simulink model "FullFMS_2025_12_15_V0_3_7"  (R2025b)
settings: Solver=ode23tb  StartTime=0.0  StopTime=inf  MaxStep=0.1  RelTol=1e-2
PreLoadFcn:
  | load("BUS_CONFIG.mat")
libraries: opcualib x8
(part 1 of 4)
settings Model: SimulationMode=accelerator  PacingRate=0.100000  Creator=guilh  LastModifiedBy=vitor
settings SolverCC: ZeroCrossControl=DisableAll

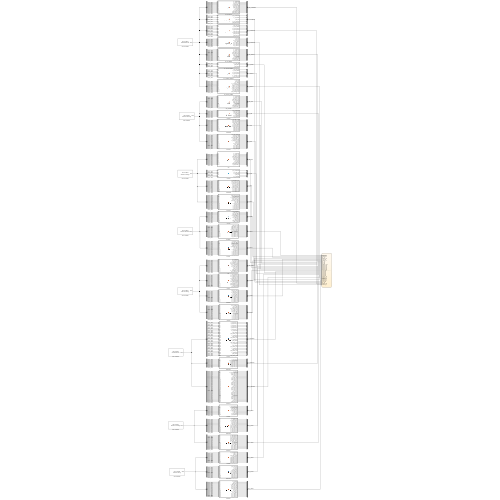
[thumbnail: Simulink's stored preview of the top-level diagram]
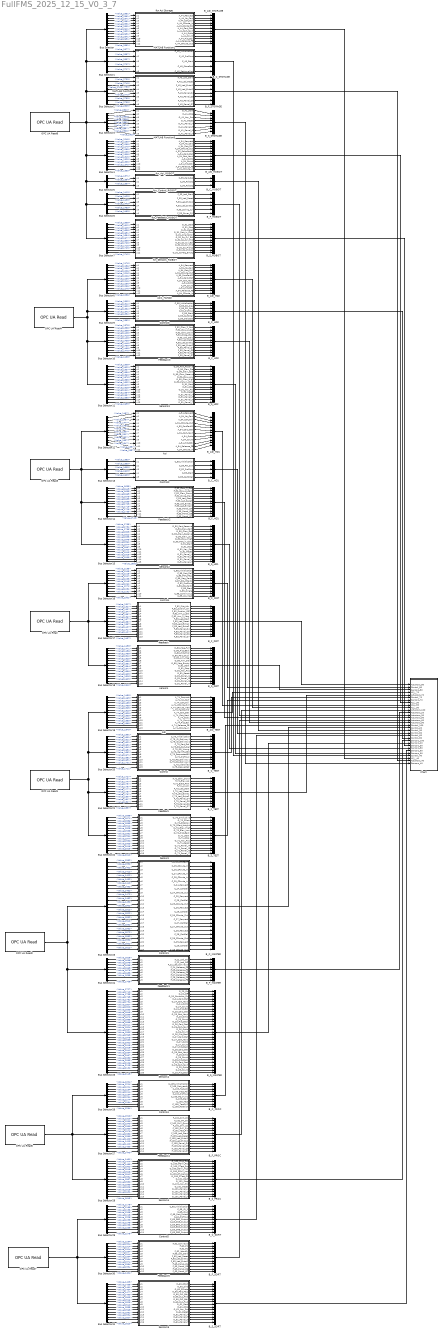
== system FullFMS_2025_12_15_V0_3_7 ==
  ASI : MATLAB Function  TreatAsAtomicUnit=on
  Asi : MATLAB Function  TreatAsAtomicUnit=on
  Asi1_HAND2 : MATLAB Function  TreatAsAtomicUnit=on
  B_ASI_HD1 : BusCreator  Inputs=12  OutDataTypeStr=Bus: B_ASI_HD1  NonVirtualBus=on
  B_ASI_HD2 : BusCreator  Inputs=12  OutDataTypeStr=Bus: B_ASI_HD2  NonVirtualBus=on
  B_ASI_ROBOT : BusCreator  Inputs=12  OutDataTypeStr=Bus: B_ASI_ROBOT  NonVirtualBus=on
  B_ASI_STORAGE : BusCreator  Inputs=12  OutDataTypeStr=Bus: B_ASI_STORAGE  NonVirtualBus=on
  B_ASI_TEST : BusCreator  Inputs=13  OutDataTypeStr=Bus: B_ASI_TEST  NonVirtualBus=on
  B_C_DIST : BusCreator  Inputs=11  OutDataTypeStr=Bus: B_C_DIST  NonVirtualBus=on
  B_C_HD1 : BusCreator  Inputs=5  OutDataTypeStr=Bus: B_C_HD1  NonVirtualBus=on
  B_C_HD2 : BusCreator  Inputs=7  OutDataTypeStr=Bus: B_C_HD2  NonVirtualBus=on
  B_C_MASTER : BusCreator  Inputs=24  OutDataTypeStr=Bus: B_C_MASTER  NonVirtualBus=on
  B_C_PROC : BusCreator  Inputs=10  OutDataTypeStr=Bus: B_C_PROC  NonVirtualBus=on
  B_C_ROBOT : BusCreator  Inputs=3  OutDataTypeStr=Bus: B_C_ROBOT  NonVirtualBus=on
  B_C_SORT : BusCreator  Inputs=11  OutDataTypeStr=Bus: B_C_SORT  NonVirtualBus=on
  B_C_STORAGE : BusCreator  Inputs=5  OutDataTypeStr=Bus: B_C_STORAGE  NonVirtualBus=on
  B_C_TEST : BusCreator  Inputs=13  OutDataTypeStr=Bus: B_C_TEST  NonVirtualBus=on
  B_F_DIST : BusCreator  Inputs=13  OutDataTypeStr=Bus: B_F_DIST  NonVirtualBus=on
  B_F_HD1 : BusCreator  Inputs=12  OutDataTypeStr=Bus: B_F_HD1  NonVirtualBus=on
  B_F_HD2 : BusCreator  Inputs=12  OutDataTypeStr=Bus: B_F_HD2  NonVirtualBus=on
  B_F_MASTER : BusCreator  Inputs=9  OutDataTypeStr=Bus: B_F_MASTER  NonVirtualBus=on
  B_F_PROC : BusCreator  Inputs=14  OutDataTypeStr=Bus: B_F_PROC  NonVirtualBus=on
  B_F_ROBOT : BusCreator  Inputs=6  OutDataTypeStr=Bus: B_F_ROBOT  NonVirtualBus=on
  B_F_SORT : BusCreator  Inputs=12  OutDataTypeStr=Bus: B_F_SORT  NonVirtualBus=on
  B_F_STORAGE : BusCreator  Inputs=8  OutDataTypeStr=Bus: B_F_STORAGE  NonVirtualBus=on
  B_F_TEST : BusCreator  Inputs=12  OutDataTypeStr=Bus: B_F_TEST  NonVirtualBus=on
  B_S_DIST : BusCreator  Inputs=15  OutDataTypeStr=Bus: B_S_DIST  NonVirtualBus=on
  B_S_HD1 : BusCreator  Inputs=15  OutDataTypeStr=Bus: B_S_HD1  NonVirtualBus=on
  B_S_HD2 : BusCreator  Inputs=15  OutDataTypeStr=Bus: B_S_HD2  NonVirtualBus=on
  B_S_MASTER : BusCreator  Inputs=33  OutDataTypeStr=Bus: B_S_MASTER  NonVirtualBus=on
  B_S_PROC : BusCreator  Inputs=15  OutDataTypeStr=Bus: B_S_PROC  NonVirtualBus=on
  B_S_ROBOT : BusCreator  Inputs=12  OutDataTypeStr=Bus: B_S_ROBOT  NonVirtualBus=on
  B_S_SORT : BusCreator  Inputs=16  OutDataTypeStr=Bus: B_S_SORT  NonVirtualBus=on
  B_S_STORAGE : BusCreator  Inputs=8  OutDataTypeStr=Bus: B_S_STORAGE  NonVirtualBus=on
  B_S_TEST : BusCreator  Inputs=15  OutDataTypeStr=Bus: B_S_TEST  NonVirtualBus=on
  Bus Selector : BusSelector  OutputSignals=Value_2551,Value_2561,Value_2571,Value_2581,Value_2591,Value_2601,Value_2611,Value_2621,Value_2631,Value_2641,Value_2651,Value_2661
  Bus Selector1 : BusSelector  OutputSignals=Value_2677,Value_2687,Value_2697,Value_2707,Value_2717
  Bus Selector10 : BusSelector  OutputSignals=Value_1378,Value_1388,Value_1398,Value_1408,Value_1418,Value_1428,Value_1438,Value_1448,Value_1458,Value_1468,Value_1478,Value_1488
  Bus Selector11 : BusSelector  OutputSignals=Value_1509,Value_1522,Value_1537,Value_1550,Value_1563,Value_1576,Value_1589,Value_1602,Value_1615,Value_1628,Value_1641,Value_1654,Value_1667,Value_1680,Value_1693
  Bus Selector12 : BusSelector  OutputSignals=Value_1457,Value_1467,Value_1477,Value_1487,Value_1497,Value_1507,Value_1517,Value_1527,Value_1537,Value_1547,Value_1557,Value_1567
  Bus Selector13 : BusSelector  OutputSignals=Value_1583,Value_1593,Value_1603,Value_1613,Value_1623
  Bus Selector14 : BusSelector  OutputSignals=Value_1639,Value_1649,Value_1659,Value_1669,Value_1679,Value_1689,Value_1699,Value_1709,Value_1719,Value_1729,Value_1739,Value_1749
  Bus Selector15 : BusSelector  OutputSignals=Value_1768,Value_1781,Value_1796,Value_1809,Value_1822,Value_1835,Value_1848,Value_1861,Value_1874,Value_1887,Value_1900,Value_1913,Value_1926,Value_1939,Value_1952
  Bus Selector16 : BusSelector  OutputSignals=Value_1195,Value_1205,Value_1215,Value_1227,Value_1239,Value_1249,Value_1261,Value_1271,Value_1281,Value_1291,Value_1301
  Bus Selector17 : BusSelector  OutputSignals=Value_1317,Value_1327,Value_1337,Value_1347,Value_1357,Value_1367,Value_1377,Value_1387,Value_1397,Value_1407,Value_1417,Value_1427,Value_1437
  Bus Selector18 : BusSelector  OutputSignals=Value_1458,Value_1471,Value_1486,Value_1499,Value_1512,Value_1525,Value_1538,Value_1551,Value_1564,Value_1577,Value_1590,Value_1603,Value_1616,Value_1629,Value_1642
  Bus Selector19 : BusSelector  OutputSignals=Value_1455,Value_1465,Value_1475,Value_1485,Value_1495,Value_1505,Value_1515,Value_1525,Value_1535,Value_1545,Value_1555,Value_1565,Value_1575
  Bus Selector2 : BusSelector  OutputSignals=Value_2733,Value_2743,Value_2753,Value_2763,Value_2773,Value_2783,Value_2793,Value_2803
  Bus Selector20 : BusSelector  OutputSignals=Value_1591,Value_1601,Value_1611,Value_1621,Value_1631,Value_1641,Value_1651,Value_1661,Value_1671,Value_1681,Value_1691,Value_1701,Value_1711
  Bus Selector21 : BusSelector  OutputSignals=Value_1727,Value_1737,Value_1747,Value_1757,Value_1767,Value_1777,Value_1787,Value_1797,Value_1807,Value_1817,Value_1827,Value_1837
  Bus Selector22 : BusSelector  OutputSignals=Value_1858,Value_1871,Value_1886,Value_1899,Value_1912,Value_1925,Value_1938,Value_1951,Value_1964,Value_1977,Value_1990,Value_2003,Value_2016,Value_2029,Value_2042
  Bus Selector23 : BusSelector  OutputSignals=Value_1382,Value_1392,Value_1402,Value_1412,Value_1422,Value_1432,Value_1442,Value_1452,Value_1462,Value_1472,Value_1482,Value_1492,Value_1502,Value_1512,Value_1522,Value_1532,Value_1542,Value_1552,Value_1562,Value_1572,Value_1582,Value_1592,Value_1602,Value_1612
  Bus Selector24 : BusSelector  OutputSignals=Value_1628,Value_1638,Value_1648,Value_1658,Value_1668,Value_1678,Value_1688,Value_1698,Value_1708
  Bus Selector25 : BusSelector  OutputSignals=Value_1727,Value_1740,Value_1755,Value_1768,Value_1781,Value_1794,Value_1807,Value_1820,Value_1833,Value_1846,Value_1859,Value_1872,Value_1885,Value_1898,Value_1911,Value_1924,Value_1937,Value_1950,Value_1963,Value_1976,Value_1989,Value_2002,Value_2015,Value_2028,Value_2041,Value_2054,Value_2067,Value_2080,Value_2093,Value_2106,Value_2119,Value_2132,Value_2145
  Bus Selector26 : BusSelector  OutputSignals=Value_1204,Value_1214,Value_1224,Value_1234,Value_1244,Value_1254,Value_1264,Value_1274,Value_1284,Value_1294
  Bus Selector27 : BusSelector  OutputSignals=Value_1310,Value_1320,Value_1330,Value_1340,Value_1350,Value_1360,Value_1370,Value_1380,Value_1390,Value_1400,Value_1410,Value_1420,Value_1430,Value_1440
  Bus Selector28 : BusSelector  OutputSignals=Value_1461,Value_1474,Value_1489,Value_1502,Value_1515,Value_1528,Value_1541,Value_1554,Value_1567,Value_1580,Value_1593,Value_1606,Value_1619,Value_1632,Value_1645
  Bus Selector29 : BusSelector  OutputSignals=Value_1178,Value_1188,Value_1198,Value_1208,Value_1218,Value_1228,Value_1238,Value_1248,Value_1258,Value_1268,Value_1278
  Bus Selector3 : BusSelector  OutputSignals=Value_2822,Value_2835,Value_2848,Value_2861,Value_2874,Value_2887,Value_2900,Value_2913
  Bus Selector30 : BusSelector  OutputSignals=Value_1294,Value_1304,Value_1314,Value_1324,Value_1334,Value_1344,Value_1354,Value_1364,Value_1374,Value_1384,Value_1394,Value_1404
  Bus Selector31 : BusSelector  OutputSignals=Value_1423,Value_1436,Value_1451,Value_1464,Value_1477,Value_1490,Value_1503,Value_1516,Value_1529,Value_1542,Value_1555,Value_1568,Value_1581,Value_1594,Value_1607,Value_1620
  Bus Selector4 : BusSelector  OutputSignals=Value_1245,Value_1255,Value_1265,Value_1275,Value_1285,Value_1295,Value_1305,Value_1315,Value_1325,Value_1335,Value_1345,Value_1355
  Bus Selector5 : BusSelector  OutputSignals=Value_1371,Value_1384,Value_1397
  Bus Selector6 : BusSelector  OutputSignals=Value_1413,Value_1423,Value_1433,Value_1443,Value_1453,Value_1463
  Bus Selector7 : BusSelector  OutputSignals=Value_1599,Value_1612,Value_1625,Value_1638,Value_1651,Value_1664,Value_1677,Value_1690,Value_1703,Value_1716,Value_1729,Value_1742
  Bus Selector8 : BusSelector  OutputSignals=Value_1176,Value_1186,Value_1196,Value_1206,Value_1216,Value_1226,Value_1236,Value_1246,Value_1256,Value_1266,Value_1276,Value_1286
  Bus Selector9 : BusSelector  OutputSignals=Value_1302,Value_1312,Value_1322,Value_1332,Value_1342,Value_1352,Value_1362
  Chart : Stateflow chart  TreatAsAtomicUnit=on
      settings: PortSchema="{\"entries\":[{\"content\":{\"sides\":[{\"content\":{\"connectorIds\":[\"In2\",\"In1\",\"In3\",\"In4\",\"In6\",\"In5\",\"In7\",\"In8\",\"In9\",\"In10\",\"In11\",\"In12\",\"In13\",\"In14\",\"In15\",\"In16\",\"In17\",\"In18\",\"In19\",\"In20\",\"In21\",\"In22\",\"In23\",\"In24\",\"In25\",\"In26\",\"In27\",\"In28\",\"In29\",\"In30\",\"In31\",\"In32\"]},\"type\":\"ConnectorPlacement.EquallySpacedRectSide\",\"uuid\":\"e54bf7d4-7c7d-41d9-a8b8-f479ac319a99\"},{\"content\":{\"side\":\"RIGHT\"},\"type\":\"ConnectorPlacement.EquallySpacedRectSide\",\"uuid\":\"d3c20706-71bd-4e26-b40f-0ee7e71b06ee\"},{\"content\":{\"side\":\"TOP\"},\"type\":\"ConnectorPlacement.EquallySpacedRectSide\",\"uuid\":\"ecfb6920-e95b-4ed8-99f9-df5ce878328e\"}]},\"type\":\"ConnectorPlacement.EquallySpacedConnector\",\"uuid\":\"2e714192-4eea-4e1a-8945-7c827feed48f\"}],\"packageUris\":[\"http://schema.mathworks.com/mf0/Connector/R2020b\"],\"version\":\"1.0\"}"
  Control : MATLAB Function  TreatAsAtomicUnit=on
  Control1 : MATLAB Function  TreatAsAtomicUnit=on
  Control2 : MATLAB Function  TreatAsAtomicUnit=on
  Control3 : MATLAB Function  TreatAsAtomicUnit=on
  Control4 : MATLAB Function  TreatAsAtomicUnit=on
  Control5 : MATLAB Function  TreatAsAtomicUnit=on
  Feedback : MATLAB Function  TreatAsAtomicUnit=on
  Feedback1 : MATLAB Function  TreatAsAtomicUnit=on
  Feedback2 : MATLAB Function  TreatAsAtomicUnit=on
  Feedback3 : MATLAB Function  TreatAsAtomicUnit=on
  Feedback4 : MATLAB Function  TreatAsAtomicUnit=on
  Feedback5 : MATLAB Function  TreatAsAtomicUnit=on
  MATLAB Function1 : MATLAB Function  TreatAsAtomicUnit=on
  MATLAB Function2 : MATLAB Function  TreatAsAtomicUnit=on
  MATLAB Function3 : MATLAB Function  TreatAsAtomicUnit=on
  OPC UA Read : opcualib/OPC UA Read  SelectedServer=AAS OPC Distribution  ServerList=AAS OPC Distribution  NodeList={ '1', 'Value', '6', '1195', '1'; '2', 'Value', '6', '1205', '1'; '3', 'Value', '6', '1215', '1'; '4', 'Value', '6', '1227', '1'; '5', 'Value', '6', '1239', '1'; '6', 'Value', '6', '1249', '1'; '7', 'Value', '6', '1261', '1'; '8', 'Value', '6', '1271', '1'; '9', 'Value', '6', '1281', '1'; '10', 'Value', '6', '1291', '1'; '11', 'Value', '6', '1301', '1'; '12', 'Value', '6', '1317', '1'; '13', 'Value', '6', '1327', '1'; '14', 'Value', '6', '1337', '1'; '15', 'Value', '6', '1347', '1'; '16', 'Value', '6', '1357', '1'; '17', 'Value', '6', '1367', '1'; '18', 'Value', '6', '1377', '1'; '19', 'Value', '6', '1387', '1'; '20', 'Value', '6', '1397', '1'; '21', 'Value', '6', '1407', '1'; '22', 'Value', '6', '1417', '1'; '23', 'Value', '6', '1427', '1'; '24', 'Value', '6', '1437', '1'; '25', 'Value', '6', '1458', '1'; '26', 'Value', '6', '1471', '1'; '27', 'Value', '6', '1486', '1'; '28', 'Value', '6', '1499', '1'; '29', 'Value', '6', '1512', '1'; '30', 'Value', '6', '1525', '1'; '31', 'Value', '6', '1538', '1'; '32', 'Value', '6', '1551', '1'; '33', 'Value', '6', '1564', '1'; '34', 'Value', '6', '1577', '1'; '35', 'Value', '6', '1590', '1'; '36', 'Value', '6', '1603', '1'; '37', 'Value', '6', '1616', '1'; '38', 'Value', '6', '1629', '1'; '39', 'Value', '6', '1642', '1' }  ShowQualityPort=off  ShowTimestampPort=off  ShowTimestampPortAs=Seconds since start  SampleTime=-1
  OPC UA Read1 : opcualib/OPC UA Read  SelectedServer=AAS OPC Testing  ServerList=AAS OPC Testing  NodeList={ '1', 'Value', '6', '1455', '1'; '2', 'Value', '6', '1465', '1'; '3', 'Value', '6', '1475', '1'; '4', 'Value', '6', '1485', '1'; '5', 'Value', '6', '1495', '1'; '6', 'Value', '6', '1505', '1'; '7', 'Value', '6', '1515', '1'; '8', 'Value', '6', '1525', '1'; '9', 'Value', '6', '1535', '1'; '10', 'Value', '6', '1545', '1'; '11', 'Value', '6', '1555', '1'; '12', 'Value', '6', '1565', '1'; '13', 'Value', '6', '1575', '1'; '14', 'Value', '6', '1591', '1'; '15', 'Value', '6', '1601', '1'; '16', 'Value', '6', '1611', '1'; '17', 'Value', '6', '1621', '1'; '18', 'Value', '6', '1631', '1'; '19', 'Value', '6', '1641', '1'; '20', 'Value', '6', '1651', '1'; '21', 'Value', '6', '1661', '1'; '22', 'Value', '6', '1671', '1'; '23', 'Value', '6', '1681', '1'; '24', 'Value', '6', '1691', '1'; '25', 'Value', '6', '1701', '1'; '26', 'Value', '6', '1711', '1'; '27', 'Value', '6', '1727', '1'; '28', 'Value', '6', '1737', '1'; '29', 'Value', '6', '1747', '1'; '30', 'Value', '6', '1757', '1'; '31', 'Value', '6', '1767', '1'; '32', 'Value', '6', '1777', '1'; '33', 'Value', '6', '1787', '1'; '34', 'Value', '6', '1797', '1'; '35', 'Value', '6', '1807', '1'; '36', 'Value', '6', '1817', '1'; '37', 'Value', '6', '1827', '1'; '38', 'Value', '6', '1837', '1'; '39', 'Value', '6', '1858', '1'; '40', 'Value', '6', '1871', '1'; '41', 'Value', '6', '1886', '1'; '42', 'Value', '6', '1899', '1'; '43', 'Value', '6', '1912', '1'; '44', 'Value', '6', '1925', '1'; '45', 'Value', '6', '1938', '1'; '46', 'Value', '6', '1951', '1'; '47', 'Value', '6', '1964', '1'; '48', 'Value', '6', '1977', '1'; '49', 'Value', '6', '1990', '1'; '50', 'Value', '6', '2003', '1'; '51', 'Value', '6', '2016', '1'; '52', 'Value', '6', '2029', '1'; '53', 'Value', '6', '2042', '1' }  ShowQualityPort=off  ShowTimestampPort=off  ShowTimestampPortAs=Seconds since start  SampleTime=-1
  OPC UA Read2 : opcualib/OPC UA Read  SelectedServer=AAS OPC Master  ServerList=AAS OPC Master  NodeList={ '1', 'Value', '6', '1382', '1'; '2', 'Value', '6', '1392', '1'; '3', 'Value', '6', '1402', '1'; '4', 'Value', '6', '1412', '1'; '5', 'Value', '6', '1422', '1'; '6', 'Value', '6', '1432', '1'; '7', 'Value', '6', '1442', '1'; '8', 'Value', '6', '1452', '1'; '9', 'Value', '6', '1462', '1'; '10', 'Value', '6', '1472', '1'; '11', 'Value', '6', '1482', '1'; '12', 'Value', '6', '1492', '1'; '13', 'Value', '6', '1502', '1'; '14', 'Value', '6', '1512', '1'; '15', 'Value', '6', '1522', '1'; '16', 'Value', '6', '1532', '1'; '17', 'Value', '6', '1542', '1'; '18', 'Value', '6', '1552', '1'; '19', 'Value', '6', '1562', '1'; '20', 'Value', '6', '1572', '1'; '21', 'Value', '6', '1582', '1'; '22', 'Value', '6', '1592', '1'; '23', 'Value', '6', '1602', '1'; '24', 'Value', '6', '1612', '1'; '25', 'Value', '6', '1628', '1'; '26', 'Value', '6', '1638', '1'; '27', 'Value', '6', '1648', '1'; '28', 'Value', '6', '1658', '1'; '29', 'Value', '6', '1668', '1'; '30', 'Value', '6', '1678', '1'; '31', 'Value', '6', '1688', '1'; '32', 'Value', '6', '1698', '1'; '33', 'Value', '6', '1708', '1'; '34', 'Value', '6', '1727', '1'; '35', 'Value', '6', '1740', '1'; '36', 'Value', '6', '1755', '1'; '37', 'Value', '6', '1768', '1'; '38', 'Value', '6', '1781', '1'; '39', 'Value', '6', '1794', '1'; '40', 'Value', '6', '1807', '1'; '41', 'Value', '6', '1820', '1'; '42', 'Value', '6', '1833', '1'; '43', 'Value', '6', '1846', '1'; '44', 'Value', '6', '1859', '1'; '45', 'Value', '6', '1872', '1'; '46', 'Value', '6', '1885', '1'; '47', 'Value', '6', '1898', '1'; '48', 'Value', '6', '1911', '1'; '49', 'Value', '6', '1924', '1'; '50', 'Value', '6', '1937', '1'; '51', 'Value', '6', '1950', '1'; '52', 'Value', '6', '1963', '1'; '53', 'Value', '6', '1976', '1'; '54', 'Value', '6', '1989', '1'; '55', 'Value', '6', '2002', '1'; '56', 'Value', '6', '2015', '1'; '57', 'Value', '6', '2028', '1'; '58', 'Value', '6', '2041', '1'; '59', 'Value', '6', '2054', '1'; '60', 'Value', '6', '2067', '1'; '61', 'Value', '6', '2080', '1'; '62', 'Value', '6', '2093', '1'; '63', 'Value', '6', '2106', '1'; '64', 'Value', '6', '2119', '1'; '65', 'Value', '6', '2132', '1'; '66', 'Value', '6', '2145', '1' }  ShowQualityPort=off  ShowTimestampPort=off  ShowTimestampPortAs=Seconds since start  SampleTime=-1
  OPC UA Read3 : opcualib/OPC UA Read  SelectedServer=AAS OPC Handling1  ServerList=AAS OPC Handling1  NodeList={ '1', 'Value', '6', '1457', '1'; '2', 'Value', '6', '1467', '1'; '3', 'Value', '6', '1477', '1'; '4', 'Value', '6', '1487', '1'; '5', 'Value', '6', '1497', '1'; '6', 'Value', '6', '1507', '1'; '7', 'Value', '6', '1517', '1'; '8', 'Value', '6', '1527', '1'; '9', 'Value', '6', '1537', '1'; '10', 'Value', '6', '1547', '1'; '11', 'Value', '6', '1557', '1'; '12', 'Value', '6', '1567', '1'; '13', 'Value', '6', '1583', '1'; '14', 'Value', '6', '1593', '1'; '15', 'Value', '6', '1603', '1'; '16', 'Value', '6', '1613', '1'; '17', 'Value', '6', '1623', '1'; '18', 'Value', '6', '1639', '1'; '19', 'Value', '6', '1649', '1'; '20', 'Value', '6', '1659', '1'; '21', 'Value', '6', '1669', '1'; '22', 'Value', '6', '1679', '1'; '23', 'Value', '6', '1689', '1'; '24', 'Value', '6', '1699', '1'; '25', 'Value', '6', '1709', '1'; '26', 'Value', '6', '1719', '1'; '27', 'Value', '6', '1729', '1'; '28', 'Value', '6', '1739', '1'; '29', 'Value', '6', '1749', '1'; '30', 'Value', '6', '1768', '1'; '31', 'Value', '6', '1781', '1'; '32', 'Value', '6', '1796', '1'; '33', 'Value', '6', '1809', '1'; '34', 'Value', '6', '1822', '1'; '35', 'Value', '6', '1835', '1'; '36', 'Value', '6', '1848', '1'; '37', 'Value', '6', '1861', '1'; '38', 'Value', '6', '1874', '1'; '39', 'Value', '6', '1887', '1'; '40', 'Value', '6', '1900', '1'; '41', 'Value', '6', '1913', '1'; '42', 'Value', '6', '1926', '1'; '43', 'Value', '6', '1939', '1'; '44', 'Value', '6', '1952', '1' }  ShowQualityPort=off  ShowTimestampPort=off  ShowTimestampPortAs=Seconds since start  SampleTime=-1
  OPC UA Read4 : opcualib/OPC UA Read  SelectedServer=AAS OPC Handling2  ServerList=AAS OPC Handling2  NodeList={ '1', 'Value', '6', '1176', '1'; '2', 'Value', '6', '1186', '1'; '3', 'Value', '6', '1196', '1'; '4', 'Value', '6', '1206', '1'; '5', 'Value', '6', '1216', '1'; '6', 'Value', '6', '1226', '1'; '7', 'Value', '6', '1236', '1'; '8', 'Value', '6', '1246', '1'; '9', 'Value', '6', '1256', '1'; '10', 'Value', '6', '1266', '1'; '11', 'Value', '6', '1276', '1'; '12', 'Value', '6', '1286', '1'; '13', 'Value', '6', '1302', '1'; '14', 'Value', '6', '1312', '1'; '15', 'Value', '6', '1322', '1'; '16', 'Value', '6', '1332', '1'; '17', 'Value', '6', '1342', '1'; '18', 'Value', '6', '1352', '1'; '19', 'Value', '6', '1362', '1'; '20', 'Value', '6', '1378', '1'; '21', 'Value', '6', '1388', '1'; '22', 'Value', '6', '1398', '1'; '23', 'Value', '6', '1408', '1'; '24', 'Value', '6', '1418', '1'; '25', 'Value', '6', '1428', '1'; '26', 'Value', '6', '1438', '1'; '27', 'Value', '6', '1448', '1'; '28', 'Value', '6', '1458', '1'; '29', 'Value', '6', '1468', '1'; '30', 'Value', '6', '1478', '1'; '31', 'Value', '6', '1488', '1'; '32', 'Value', '6', '1509', '1'; '33', 'Value', '6', '1522', '1'; '34', 'Value', '6', '1537', '1'; '35', 'Value', '6', '1550', '1'; '36', 'Value', '6', '1563', '1'; '37', 'Value', '6', '1576', '1'; '38', 'Value', '6', '1589', '1'; '39', 'Value', '6', '1602', '1'; '40', 'Value', '6', '1615', '1'; '41', 'Value', '6', '1628', '1'; '42', 'Value', '6', '1641', '1'; '43', 'Value', '6', '1654', '1'; '44', 'Value', '6', '1667', '1'; '45', 'Value', '6', '1680', '1'; '46', 'Value', '6', '1693', '1' }  ShowQualityPort=off  ShowTimestampPort=off  ShowTimestampPortAs=Seconds since start  SampleTime=-1
  OPC UA Read5 : opcualib/OPC UA Read  SelectedServer=AAS OPC Processing  ServerList=AAS OPC Processing  NodeList={ '1', 'Value', '6', '1204', '1'; '2', 'Value', '6', '1214', '1'; '3', 'Value', '6', '1224', '1'; '4', 'Value', '6', '1234', '1'; '5', 'Value', '6', '1244', '1'; '6', 'Value', '6', '1254', '1'; '7', 'Value', '6', '1264', '1'; '8', 'Value', '6', '1274', '1'; '9', 'Value', '6', '1284', '1'; '10', 'Value', '6', '1294', '1'; '11', 'Value', '6', '1310', '1'; '12', 'Value', '6', '1320', '1'; '13', 'Value', '6', '1330', '1'; '14', 'Value', '6', '1340', '1'; '15', 'Value', '6', '1350', '1'; '16', 'Value', '6', '1360', '1'; '17', 'Value', '6', '1370', '1'; '18', 'Value', '6', '1380', '1'; '19', 'Value', '6', '1390', '1'; '20', 'Value', '6', '1400', '1'; '21', 'Value', '6', '1410', '1'; '22', 'Value', '6', '1420', '1'; '23', 'Value', '6', '1430', '1'; '24', 'Value', '6', '1440', '1'; '25', 'Value', '6', '1461', '1'; '26', 'Value', '6', '1474', '1'; '27', 'Value', '6', '1489', '1'; '28', 'Value', '6', '1502', '1'; '29', 'Value', '6', '1515', '1'; '30', 'Value', '6', '1528', '1'; '31', 'Value', '6', '1541', '1'; '32', 'Value', '6', '1554', '1'; '33', 'Value', '6', '1567', '1'; '34', 'Value', '6', '1580', '1'; '35', 'Value', '6', '1593', '1'; '36', 'Value', '6', '1606', '1'; '37', 'Value', '6', '1619', '1'; '38', 'Value', '6', '1632', '1'; '39', 'Value', '6', '1645', '1' }  ShowQualityPort=off  ShowTimestampPort=off  ShowTimestampPortAs=Seconds since start  SampleTime=-1
  OPC UA Read6 : opcualib/OPC UA Read  SelectedServer=Node-RED OPCUA  ServerList=Node-RED OPCUA  NodeList={ '1', 'Value', '6', '2551', '1'; '2', 'Value', '6', '2561', '1'; '3', 'Value', '6', '2571', '1'; '4', 'Value', '6', '2581', '1'; '5', 'Value', '6', '2591', '1'; '6', 'Value', '6', '2601', '1'; '7', 'Value', '6', '2611', '1'; '8', 'Value', '6', '2621', '1'; '9', 'Value', '6', '2631', '1'; '10', 'Value', '6', '2641', '1'; '11', 'Value', '6', '2651', '1'; '12', 'Value', '6', '2661', '1'; '13', 'Value', '6', '2677', '1'; '14', 'Value', '6', '2687', '1'; '15', 'Value', '6', '2697', '1'; '16', 'Value', '6', '2707', '1'; '17', 'Value', '6', '2717', '1'; '18', 'Value', '6', '2733', '1'; '19', 'Value', '6', '2743', '1'; '20', 'Value', '6', '2753', '1'; '21', 'Value', '6', '2763', '1'; '22', 'Value', '6', '2773', '1'; '23', 'Value', '6', '2783', '1'; '24', 'Value', '6', '2793', '1'; '25', 'Value', '6', '2803', '1'; '26', 'Value', '6', '2822', '1'; '27', 'Value', '6', '2835', '1'; '28', 'Value', '6', '2848', '1'; '29', 'Value', '6', '2861', '1'; '30', 'Value', '6', '2874', '1'; '31', 'Value', '6', '2887', '1'; '32', 'Value', '6', '2900', '1'; '33', 'Value', '6', '2913', '1'; '34', 'Value', '6', '1245', '1'; '35', 'Value', '6', '1255', '1'; '36', 'Value', '6', '1265', '1'; '37', 'Value', '6', '1275', '1'; '38', 'Value', '6', '1285', '1'; '39', 'Value', '6', '1295', '1'; '40', 'Value', '6', '1305', '1'; '41', 'Value', '6', '1315', '1'; '42', 'Value', '6', '1325', '1'; '43', 'Value', '6', '1335', '1'; '44', 'Value', '6', '1345', '1'; '45', 'Value', '6', '1355', '1'; '46', 'Value', '6', '1371', '1'; '47', 'Value', '6', '1384', '1'; '48', 'Value', '6', '1397', '1'; '49', 'Value', '6', '1413', '1'; '50', 'Value', '6', '1423', '1'; '51', 'Value', '6', '1433', '1'; '52', 'Value', '6', '1443', '1'; '53', 'Value', '6', '1453', '1'; '54', 'Value', '6', '1463', '1'; '55', 'Value', '6', '1599', '1'; '56', 'Value', '6', '1612', '1'; '57', 'Value', '6', '1625', '1'; '58', 'Value', '6', '1638', '1'; '59', 'Value', '6', '1651', '1'; '60', 'Value', '6', '1664', '1'; '61', 'Value', '6', '1677', '1'; '62', 'Value', '6', '1690', '1'; '63', 'Value', '6', '1703', '1'; '64', 'Value', '6', '1716', '1'; '65', 'Value', '6', '1729', '1'; '66', 'Value', '6', '1742', '1' }  ShowQualityPort=off  ShowTimestampPort=off  ShowTimestampPortAs=Seconds since start  SampleTime=-1
  OPC UA Read7 : opcualib/OPC UA Read  SelectedServer=AAS OPC Sorting  ServerList=AAS OPC Sorting  NodeList={ '1', 'Value', '6', '1178', '1'; '2', 'Value', '6', '1188', '1'; '3', 'Value', '6', '1198', '1'; '4', 'Value', '6', '1208', '1'; '5', 'Value', '6', '1218', '1'; '6', 'Value', '6', '1228', '1'; '7', 'Value', '6', '1238', '1'; '8', 'Value', '6', '1248', '1'; '9', 'Value', '6', '1258', '1'; '10', 'Value', '6', '1268', '1'; '11', 'Value', '6', '1278', '1'; '12', 'Value', '6', '1294', '1'; '13', 'Value', '6', '1304', '1'; '14', 'Value', '6', '1314', '1'; '15', 'Value', '6', '1324', '1'; '16', 'Value', '6', '1334', '1'; '17', 'Value', '6', '1344', '1'; '18', 'Value', '6', '1354', '1'; '19', 'Value', '6', '1364', '1'; '20', 'Value', '6', '1374', '1'; '21', 'Value', '6', '1384', '1'; '22', 'Value', '6', '1394', '1'; '23', 'Value', '6', '1404', '1'; '24', 'Value', '6', '1423', '1'; '25', 'Value', '6', '1436', '1'; '26', 'Value', '6', '1451', '1'; '27', 'Value', '6', '1464', '1'; '28', 'Value', '6', '1477', '1'; '29', 'Value', '6', '1490', '1'; '30', 'Value', '6', '1503', '1'; '31', 'Value', '6', '1516', '1'; '32', 'Value', '6', '1529', '1'; '33', 'Value', '6', '1542', '1'; '34', 'Value', '6', '1555', '1'; '35', 'Value', '6', '1568', '1'; '36', 'Value', '6', '1581', '1'; '37', 'Value', '6', '1594', '1'; '38', 'Value', '6', '1607', '1'; '39', 'Value', '6', '1620', '1' }  ShowQualityPort=off  ShowTimestampPort=off  ShowTimestampPortAs=Seconds since start  SampleTime=-1
  Sensors : MATLAB Function  TreatAsAtomicUnit=on
  Sensors1 : MATLAB Function  TreatAsAtomicUnit=on
  Sensors2 : MATLAB Function  TreatAsAtomicUnit=on
  Sensors3 : MATLAB Function  TreatAsAtomicUnit=on
  Sensors4 : MATLAB Function  TreatAsAtomicUnit=on
  Sensors5 : MATLAB Function  TreatAsAtomicUnit=on
  controls : MATLAB Function  TreatAsAtomicUnit=on
  fcn Asi Storage : MATLAB Function  TreatAsAtomicUnit=on
  fcn_Asi_ROBOT : MATLAB Function  TreatAsAtomicUnit=on
  fcn_Control_ROBOT : MATLAB Function  TreatAsAtomicUnit=on
  fcn_Feedback_ROBOT : MATLAB Function  TreatAsAtomicUnit=on
  fcn_Sensors_ROBOT : MATLAB Function  TreatAsAtomicUnit=on
  feedback : MATLAB Function  TreatAsAtomicUnit=on
  sensors : MATLAB Function  TreatAsAtomicUnit=on
  wires:
  feedback/1(F_82_Pist_Adv) -> B_F_DIST/1
  feedback/2(F_82_Suction_On) -> B_F_DIST/2
  feedback/3(F_82_Suction_Off) -> B_F_DIST/3
  feedback/4(F_82_Arm_2_Del) -> B_F_DIST/4
  feedback/5(F_82_Arm_2_Mag) -> B_F_DIST/5
  feedback/6(F_83_Led_Start) -> B_F_DIST/6
  feedback/7(F_83_Led_Reset) -> B_F_DIST/7
  feedback/8(F_83_Led_Extra1) -> B_F_DIST/8
  feedback/9(F_83_Led_Extra2) -> B_F_DIST/9
  feedback/10(F_83_Panel_O4) -> B_F_DIST/10
  feedback/11(F_83_Panel_O5) -> B_F_DIST/11
  feedback/12(F_83_Panel_O6) -> B_F_DIST/12
  feedback/13(F_83_Panel_O7) -> B_F_DIST/13
  sensors/1(O_80_Mag_Full) -> B_S_DIST/1
  sensors/2(O_80_Pist_Back) -> B_S_DIST/2
  sensors/3(O_80_Pist_Fwd) -> B_S_DIST/3
  sensors/4(O_80_Part_Stuck) -> B_S_DIST/4
  sensors/5(O_80_Arm_Mag) -> B_S_DIST/5
  sensors/6(O_80_Arm_Del) -> B_S_DIST/6
  sensors/7(O_80_Mag_Empty) -> B_S_DIST/7
  sensors/8(O_81_Start) -> B_S_DIST/8
  sensors/9(O_81_Stop) -> B_S_DIST/9
  sensors/10(O_81_Key_Pos) -> B_S_DIST/10
  sensors/11(O_81_Reset) -> B_S_DIST/11
  sensors/12(O_81_Panel_I4) -> B_S_DIST/12
  sensors/13(O_81_Panel_I5) -> B_S_DIST/13
  sensors/14(O_81_Panel_I6) -> B_S_DIST/14
  sensors/15(O_81_Panel_I7) -> B_S_DIST/15
  ASI/1(A_74_Request) -> B_ASI_TEST/1
  ASI/2(A_74_No_Cart) -> B_ASI_TEST/2
  ASI/3(A_74_Cart_Full) -> B_ASI_TEST/3
  ASI/4(A_74_CRoute_Out) -> B_ASI_TEST/4
  ASI/5(A_74_CRoute_In80) -> B_ASI_TEST/5
  ASI/6(A_73_TestCartID) -> B_ASI_TEST/6
  ASI/7(A_74_Cart_Stat) -> B_ASI_TEST/7
  ASI/8(A_74_Cart_Next) -> B_ASI_TEST/8
  ASI/9(A_74_Optic) -> B_ASI_TEST/9
  ASI/10(A_74_Count) -> B_ASI_TEST/10
  ASI/11(A_74_Pist_Bck) -> B_ASI_TEST/11
  ASI/12(A_74_Release_FB) -> B_ASI_TEST/12
  ASI/13(A_74_CRoute_In) -> B_ASI_TEST/13
  Control/1(C_75_Initialization) -> B_C_TEST/1
  Control/2(C_75_ID_Delivery1) -> B_C_TEST/2
  Control/3(C_75_ID_Delivery2) -> B_C_TEST/3
  Control/4(C_75_Part_Del) -> B_C_TEST/4
  Control/5(C_75_RQ_Part_Del) -> B_C_TEST/5
  Control/6(C_75_RQ_Wrong) -> B_C_TEST/6
  Control/7(C_75_Identified80) -> B_C_TEST/7
  Control/8(C_75_Requested80) -> B_C_TEST/8
  Control/9(C_72_Profibus) -> B_C_TEST/9
  Control/10(C_75_RQ_Delivery1) -> B_C_TEST/10
  Control/11(C_75_RQ_Delivery2) -> B_C_TEST/11
  Control/12(C_75_Identified) -> B_C_TEST/12
  Control/13(C_75_Requested) -> B_C_TEST/13
  Feedback/1(F_72_Elev_Down) -> B_F_TEST/1
  Feedback/2(F_72_Elev_Up) -> B_F_TEST/2
  Feedback/3(F_72_Eject_Part) -> B_F_TEST/3
  Feedback/4(F_72_Air_On) -> B_F_TEST/4
  Feedback/5(F_73_Led_Start) -> B_F_TEST/5
  Feedback/6(F_73_Led_Reset) -> B_F_TEST/6
  Feedback/7(F_73_Led_Extra1) -> B_F_TEST/7
  Feedback/8(F_73_Led_Extra2) -> B_F_TEST/8
  Feedback/9(F_73_Panel_O4) -> B_F_TEST/9
  Feedback/10(F_73_Panel_O5) -> B_F_TEST/10
  Feedback/11(F_73_Panel_O6) -> B_F_TEST/11
  Feedback/12(F_73_Panel_O7) -> B_F_TEST/12
  Sensors/1(O_70_SInductive) -> B_S_TEST/1
  Sensors/2(O_70_SPart) -> B_S_TEST/2
  Sensors/3(O_70_SStation) -> B_S_TEST/3
  Sensors/4(O_70_SPart_Height) -> B_S_TEST/4
  Sensors/5(O_70_Elev_High) -> B_S_TEST/5
  Sensors/6(O_70_Elev_Low) -> B_S_TEST/6
  Sensors/7(O_70_Pist_Back) -> B_S_TEST/7
  Sensors/8(O_71_Start) -> B_S_TEST/8
  Sensors/9(O_71_Stop) -> B_S_TEST/9
  Sensors/10(O_71_Key_Pos) -> B_S_TEST/10
  Sensors/11(O_71_Reset) -> B_S_TEST/11
  Sensors/12(O_71_Panel_I4) -> B_S_TEST/12
  Sensors/13(O_71_Panel_I5) -> B_S_TEST/13
  Sensors/14(O_71_Panel_I6) -> B_S_TEST/14
  Sensors/15(O_71_Panel_I7) -> B_S_TEST/15
  B_C_DIST/1 -> Chart/1(Control_80)
  B_F_DIST/1 -> Chart/2(Actuators_80)
  B_S_DIST/1 -> Chart/3(Sensors_80)
  B_S_TEST/1 -> Chart/7(Sensors_70)
  B_F_TEST/1 -> Chart/6(Actuators_70)
  B_C_TEST/1 -> Chart/5(Control_70)
  B_ASI_TEST/1 -> Chart/4(AS_i_70)
  Control1/1(C_24_CRoute_In) -> B_C_MASTER/1
  Control1/2(C_25_CRoute_In) -> B_C_MASTER/2
  Control1/3(C_26_CRoute_In) -> B_C_MASTER/3
  Control1/4(C_27_CRoute_In) -> B_C_MASTER/4
  Control1/5(C_28_CRoute_In) -> B_C_MASTER/5
  Control1/6(C_29_CRoute_In) -> B_C_MASTER/6
  Control1/7(C_24_Request) -> B_C_MASTER/7
  Control1/8(C_24_CartDel) -> B_C_MASTER/8
  Control1/9(C_24_CRoute_Out) -> B_C_MASTER/9
  Control1/10(C_25_Request) -> B_C_MASTER/10
  Control1/11(C_25_CartDel) -> B_C_MASTER/11
  Control1/12(C_25_CRoute_Out) -> B_C_MASTER/12
  Control1/13(C_26_Request) -> B_C_MASTER/13
  Control1/14(C_26_CartDel) -> B_C_MASTER/14
  Control1/15(C_26_CRoute_Out) -> B_C_MASTER/15
  Control1/16(C_27_Request) -> B_C_MASTER/16
  Control1/17(C_27_CartDel) -> B_C_MASTER/17
  Control1/18(C_27_CRoute_Out) -> B_C_MASTER/18
  Control1/19(C_28_Request) -> B_C_MASTER/19
  Control1/20(C_28_CartDel) -> B_C_MASTER/20
  Control1/21(C_28_CRoute_Out) -> B_C_MASTER/21
  Control1/22(C_29_Request) -> B_C_MASTER/22
  Control1/23(C_29_CartDel) -> B_C_MASTER/23
  Control1/24(C_29_CRoute_Out) -> B_C_MASTER/24
  Feedback1/1(F_22_Led_On) -> B_F_MASTER/1
  Feedback1/2(F_22_Led_Off) -> B_F_MASTER/2
  Feedback1/3(F_22_Led_Conveyor) -> B_F_MASTER/3
  Feedback1/4(F_24_Release_FB) -> B_F_MASTER/4
  Feedback1/5(F_25_Release_FB) -> B_F_MASTER/5
  Feedback1/6(F_26_Release_FB) -> B_F_MASTER/6
  Feedback1/7(F_27_Release_FB) -> B_F_MASTER/7
  Feedback1/8(F_28_Release_FB) -> B_F_MASTER/8
  Feedback1/9(F_29_Release_FB) -> B_F_MASTER/9
  Sensors1/1(O_20_On) -> B_S_MASTER/1
  Sensors1/2(O_20_Off) -> B_S_MASTER/2
  Sensors1/3(O_20_Controler_On) -> B_S_MASTER/3
  Sensors1/4(O_24_Cart_Stat) -> B_S_MASTER/4
  Sensors1/5(O_24_Cart_Next) -> B_S_MASTER/5
  Sensors1/6(O_24_Optic) -> B_S_MASTER/6
  Sensors1/7(O_24_Count) -> B_S_MASTER/7
  Sensors1/8(O_24_Pist_Bck) -> B_S_MASTER/8
  Sensors1/9(O_25_Cart_Stat) -> B_S_MASTER/9
  Sensors1/10(O_25_Cart_Next) -> B_S_MASTER/10
  Sensors1/11(O_25_Optic) -> B_S_MASTER/11
  Sensors1/12(O_25_Count) -> B_S_MASTER/12
  Sensors1/13(O_25_Pist_Back) -> B_S_MASTER/13
  Sensors1/14(O_26_Cart_Stat) -> B_S_MASTER/14
  Sensors1/15(O_26_Cart_Next) -> B_S_MASTER/15
  Sensors1/16(O_26_Optic) -> B_S_MASTER/16
  Sensors1/17(O_26_Count) -> B_S_MASTER/17
  Sensors1/18(O_26_Pist_Back) -> B_S_MASTER/18
  Sensors1/19(O_27_Cart_Stat) -> B_S_MASTER/19
  Sensors1/20(O_27_Cart_Next) -> B_S_MASTER/20
  Sensors1/21(O_27_Optic) -> B_S_MASTER/21
  Sensors1/22(O_27_Count) -> B_S_MASTER/22
  Sensors1/23(O_27_Pist_Back) -> B_S_MASTER/23
  Sensors1/24(O_28_Cart_Stat) -> B_S_MASTER/24
  Sensors1/25(O_28_Cart_Next) -> B_S_MASTER/25
  Sensors1/26(O_28_Optic) -> B_S_MASTER/26
  Sensors1/27(O_28_Count) -> B_S_MASTER/27
  Sensors1/28(O_28_Pist_Back) -> B_S_MASTER/28
  Sensors1/29(O_29_Cart_Stat) -> B_S_MASTER/29
  Sensors1/30(O_29_Cart_Next) -> B_S_MASTER/30
  Sensors1/31(O_29_Optic) -> B_S_MASTER/31
  Sensors1/32(O_29_Count) -> B_S_MASTER/32
  Sensors1/33(O_29_Pist_Back) -> B_S_MASTER/33
  B_C_MASTER/1 -> Chart/18(Control_20)
  B_F_MASTER/1 -> Chart/12(Actuators_20)
  B_S_MASTER/1 -> Chart/24(Sensors_20)
  Sensors2/1(O_50_Part_Reserve) -> B_S_HD1/1
  Sensors2/2(O_50_Claw_Cart) -> B_S_HD1/2
  Sensors2/3(O_50_Claw_Del) -> B_S_HD1/3
  Sensors2/4(O_50_Claw_Reserve) -> B_S_HD1/4
  Sensors2/5(O_50_Claw_Low) -> B_S_HD1/5
  Sensors2/6(O_50_Claw_High) -> B_S_HD1/6
  Sensors2/7(O_50_Part_in_Claw) -> B_S_HD1/7
  Sensors2/8(O_51_Start) -> B_S_HD1/8
  Sensors2/9(O_51_Stop) -> B_S_HD1/9
  Sensors2/10(O_51_Key_Pos) -> B_S_HD1/10
  Sensors2/11(O_51_Reset) -> B_S_HD1/11
  Sensors2/12(O_51_Panel_I4) -> B_S_HD1/12
  Sensors2/13(O_51_Panel_I5) -> B_S_HD1/13
  Sensors2/14(O_51_Panel_I6) -> B_S_HD1/14
  Sensors2/15(O_51_Panel_I7) -> B_S_HD1/15
  Feedback2/1(F_52_Claw_2_Del) -> B_F_HD1/1
  Feedback2/2(F_52_Claw_2_Cart) -> B_F_HD1/2
  Feedback2/3(F_52_Claw_Down) -> B_F_HD1/3
  Feedback2/4(F_52_Close_Claw) -> B_F_HD1/4
  Feedback2/5(F_53_Led_Start) -> B_F_HD1/5
  Feedback2/6(F_53_Led_Reset) -> B_F_HD1/6
  Feedback2/7(F_53_Led_Extra1) -> B_F_HD1/7
  Feedback2/8(F_53_Led_Extra2) -> B_F_HD1/8
  Feedback2/9(F_53_Panel_O4) -> B_F_HD1/9
  Feedback2/10(F_53_Panel_O5) -> B_F_HD1/10
  Feedback2/11(F_53_Panel_O6) -> B_F_HD1/11
  Feedback2/12(F_53_Panel_O7) -> B_F_HD1/12
  Control2/1(C_55_Initialization) -> B_C_HD1/1
  Control2/2(C_55_PD_Sort) -> B_C_HD1/2
  Control2/3(C_52_Profibus) -> B_C_HD1/3
  Control2/4(C_55_Start) -> B_C_HD1/4
  Control2/5(C_55_Cart2Del) -> B_C_HD1/5
  B_ASI_HD1/1 -> Chart/9(AS_i_50)
  B_C_HD1/1 -> Chart/20(Control_50)
  B_F_HD1/1 -> Chart/14(Actuators_50)
  B_S_HD1/1 -> Chart/26(Sensors_50)
  Asi1_HAND2/1(A_94_Request) -> B_ASI_HD2/1
  Asi1_HAND2/2(A_94_No_Cart) -> B_ASI_HD2/2
  Asi1_HAND2/3(A_94_Cart_Full) -> B_ASI_HD2/3
  Asi1_HAND2/4(A_94_CRoute_Out) -> B_ASI_HD2/4
  Asi1_HAND2/5(A_93_ProcCartID) -> B_ASI_HD2/5
  Asi1_HAND2/6(A_94_Cart_Stat) -> B_ASI_HD2/6
  Asi1_HAND2/7(A_94_Cart_Next) -> B_ASI_HD2/7
  Asi1_HAND2/8(A_94_Optic) -> B_ASI_HD2/8
  Asi1_HAND2/9(A_94_Count) -> B_ASI_HD2/9
  Asi1_HAND2/10(A_94_Pist_Bck) -> B_ASI_HD2/10
  Asi1_HAND2/11(A_94_Release_FB) -> B_ASI_HD2/11
  Asi1_HAND2/12(A_94_CRoute_In) -> B_ASI_HD2/12
  Control3/1(C_95_Initialization) -> B_C_HD2/1
  Control3/2(C_95_PD_Proc) -> B_C_HD2/2
  Control3/3(C_95_PD_Cart) -> B_C_HD2/3
  Control3/4(C_92_Profibus) -> B_C_HD2/4
  Control3/5(C_95_Start) -> B_C_HD2/5
  Control3/6(C_95_Cart2Del) -> B_C_HD2/6
  Control3/7(C_95_Del2Cart) -> B_C_HD2/7
  Feedback3/1(F_92_Claw_2_Cart) -> B_F_HD2/1
  Feedback3/2(F_92_Claw_2_Del) -> B_F_HD2/2
  Feedback3/3(F_92_Claw_Down) -> B_F_HD2/3
  Feedback3/4(F_92_Close_Claw) -> B_F_HD2/4
  Feedback3/5(F_93_Led_Start) -> B_F_HD2/5
  Feedback3/6(F_93_Led_Reset) -> B_F_HD2/6
  Feedback3/7(F_93_Led_Extra1) -> B_F_HD2/7
  Feedback3/8(F_93_Led_Extra2) -> B_F_HD2/8
  Feedback3/9(F_93_Panel_O4) -> B_F_HD2/9
  Feedback3/10(F_93_Panel_O5) -> B_F_HD2/10
  Feedback3/11(F_93_Panel_O6) -> B_F_HD2/11
  Feedback3/12(F_93_Panel_O7) -> B_F_HD2/12
  Sensors3/1(O_90_Part_Reserve) -> B_S_HD2/1
  Sensors3/2(O_90_Claw_Del) -> B_S_HD2/2
  Sensors3/3(O_90_Claw_Cart) -> B_S_HD2/3
  Sensors3/4(O_90_Claw_Reserve) -> B_S_HD2/4
  Sensors3/5(O_90_Claw_Low) -> B_S_HD2/5
  Sensors3/6(O_90_Claw_High) -> B_S_HD2/6
  Sensors3/7(O_90_Part_in_Claw) -> B_S_HD2/7
  Sensors3/8(O_91_Start) -> B_S_HD2/8
  Sensors3/9(O_91_Stop) -> B_S_HD2/9
  Sensors3/10(O_91_Key_Pos) -> B_S_HD2/10
  Sensors3/11(O_91_Reset) -> B_S_HD2/11
  Sensors3/12(O_91_Panel_I4) -> B_S_HD2/12
  Sensors3/13(O_91_Panel_I5) -> B_S_HD2/13
  Sensors3/14(O_91_Panel_I6) -> B_S_HD2/14
  Sensors3/15(O_91_Panel_I7) -> B_S_HD2/15
  B_ASI_HD2/1 -> Chart/10(AS_i_90)
  B_C_HD2/1 -> Chart/22(Control_90)
  B_F_HD2/1 -> Chart/16(Actuators_90)
  B_S_HD2/1 -> Chart/28(Sensors_90)
  Sensors4/1(O_100_PInit_Pos) -> B_S_PROC/1
  Sensors4/2(O_100_PDrill_Pos) -> B_S_PROC/2
  Sensors4/3(O_100_PTest_Pos) -> B_S_PROC/3
  Sensors4/4(O_100_SDrill_High) -> B_S_PROC/4
  Sensors4/5(O_100_SDrill_Low) -> B_S_PROC/5
  Sensors4/6(O_100_RT_Sensor) -> B_S_PROC/6
  Sensors4/7(O_100_PTest_Ok) -> B_S_PROC/7
  Sensors4/8(O_101_Start) -> B_S_PROC/8
  Sensors4/9(O_101_Stop) -> B_S_PROC/9
  Sensors4/10(O_101_Key_Pos) -> B_S_PROC/10
  Sensors4/11(O_101_Reset) -> B_S_PROC/11
  Sensors4/12(O_101_Panel_I4) -> B_S_PROC/12
  Sensors4/13(O_101_Panel_I5) -> B_S_PROC/13
  Sensors4/14(O_101_Panel_I6) -> B_S_PROC/14
  Sensors4/15(O_101_Panel_I7) -> B_S_PROC/15
  Control4/1(C_105_Initialization) -> B_C_PROC/1
  Control4/2(C_105_Part_ready) -> B_C_PROC/2
  Control4/3(C_105_Test_Ok) -> B_C_PROC/3
  Control4/4(C_105_Test_Fail) -> B_C_PROC/4
  Control4/5(C_102_Profibus) -> B_C_PROC/5
  Control4/6(C_103_RQ_Turns) -> B_C_PROC/6
  Control4/7(C_105_Start) -> B_C_PROC/7
  Control4/8(C_105_Test) -> B_C_PROC/8
  Control4/9(C_105_TestDrill) -> B_C_PROC/9
  Control4/10(C_105_Rotation) -> B_C_PROC/10
  Feedback4/1(F_102_Drill_On) -> B_F_PROC/1
  Feedback4/2(F_102_RT_On) -> B_F_PROC/2
  Feedback4/3(F_102_Drill_Down) -> B_F_PROC/3
  Feedback4/4(F_102_Drill_Up) -> B_F_PROC/4
  Feedback4/5(F_102_Drill_Pin) -> B_F_PROC/5
  Feedback4/6(F_102_Test_Pin) -> B_F_PROC/6
  Feedback4/7(F_103_Led_Start) -> B_F_PROC/7
  Feedback4/8(F_103_Led_Reset) -> B_F_PROC/8
  Feedback4/9(F_103_Led_Extra1) -> B_F_PROC/9
  Feedback4/10(F_103_Led_Extra2) -> B_F_PROC/10
  Feedback4/11(F_103_Panel_O4) -> B_F_PROC/11
  Feedback4/12(F_103_Panel_O5) -> B_F_PROC/12
  Feedback4/13(F_103_Panel_O6) -> B_F_PROC/13
  Feedback4/14(F_103_Panel_O7) -> B_F_PROC/14
  B_C_PROC/1 -> Chart/17(Control_100)
  B_F_PROC/1 -> Chart/11(Actuators_100)
  B_S_PROC/1 -> Chart/23(Sensors_100)
  fcn_Asi_ROBOT/1(A_34_Request) -> B_ASI_ROBOT/1
  fcn_Asi_ROBOT/2(A_34_No_Cart) -> B_ASI_ROBOT/2
  fcn_Asi_ROBOT/3(A_34_Cart_Full) -> B_ASI_ROBOT/3
  fcn_Asi_ROBOT/4(A_34_CRoute_Out) -> B_ASI_ROBOT/4
  fcn_Asi_ROBOT/5(A_32_RoboCartID) -> B_ASI_ROBOT/5
  fcn_Asi_ROBOT/6(A_34_Cart_Stat) -> B_ASI_ROBOT/6
  fcn_Asi_ROBOT/7(A_34_Cart_Next) -> B_ASI_ROBOT/7
  fcn_Asi_ROBOT/8(A_34_Optic) -> B_ASI_ROBOT/8
  fcn_Asi_ROBOT/9(A_34_Count) -> B_ASI_ROBOT/9
  fcn_Asi_ROBOT/10(A_34_Pist_Bck) -> B_ASI_ROBOT/10
  fcn_Asi_ROBOT/11(A_34_Release_FB) -> B_ASI_ROBOT/11
  fcn_Asi_ROBOT/12(A_34_CRoute_In) -> B_ASI_ROBOT/12
  fcn_Feedback_ROBOT/1(F_33_Led_Start) -> B_F_ROBOT/1
  fcn_Feedback_ROBOT/2(F_33_Led_Reset) -> B_F_ROBOT/2
  fcn_Feedback_ROBOT/3(F_33_Led_Extra1) -> B_F_ROBOT/3
  fcn_Feedback_ROBOT/4(F_33_Led_Extra2) -> B_F_ROBOT/4
  fcn_Feedback_ROBOT/5(F_33_Spring_Cyl) -> B_F_ROBOT/5
  fcn_Feedback_ROBOT/6(F_33_Cover_Cyl) -> B_F_ROBOT/6
  fcn_Sensors_ROBOT/1(O_31_Start) -> B_S_ROBOT/1
  fcn_Sensors_ROBOT/2(O_31_Stop) -> B_S_ROBOT/2
  fcn_Sensors_ROBOT/3(O_31_Reset) -> B_S_ROBOT/3
  fcn_Sensors_ROBOT/4(O_31_Part_in_Claw) -> B_S_ROBOT/4
  fcn_Sensors_ROBOT/5(O_31_Orientation) -> B_S_ROBOT/5
  fcn_Sensors_ROBOT/6(O_32_Sp_Cyl_Bck) -> B_S_ROBOT/6
  fcn_Sensors_ROBOT/7(O_32_Sp_Cyl_Fwd) -> B_S_ROBOT/7
  fcn_Sensors_ROBOT/8(O_32_Co_Cyl_Bck) -> B_S_ROBOT/8
  fcn_Sensors_ROBOT/9(O_32_Co_Cyl_Fwd) -> B_S_ROBOT/9
  fcn_Sensors_ROBOT/10(O_32_Sp_PickUp) -> B_S_ROBOT/10
  fcn_Sensors_ROBOT/11(O_32_Co_PickUp) -> B_S_ROBOT/11
  fcn_Sensors_ROBOT/12(O_32_CoMag_Empty) -> B_S_ROBOT/12
  B_ASI_ROBOT/1 -> Chart/8(AS_i_30)
  B_C_ROBOT/1 -> Chart/19(Control_30)
  B_F_ROBOT/1 -> Chart/13(Actuators_30)
  B_S_ROBOT/1 -> Chart/25(Sensors_30)
  Control5/1(C_65_Initialization) -> B_C_SORT/1
  Control5/2(C_65_ID_1) -> B_C_SORT/2
  Control5/3(C_65_ID_2) -> B_C_SORT/3
  Control5/4(C_65_Part_Sorted) -> B_C_SORT/4
  Control5/5(C_62_Profibus) -> B_C_SORT/5
  Control5/6(C_65_RBS_Output) -> B_C_SORT/6
  Control5/7(C_65_RSB_Output) -> B_C_SORT/7
  Control5/8(C_65_BRS_Output) -> B_C_SORT/8
  Control5/9(C_65_BSR_Output) -> B_C_SORT/9
  Control5/10(C_65_SRB_Output) -> B_C_SORT/10
  Control5/11(C_65_SBR_Output) -> B_C_SORT/11
  Feedback5/1(F_62_Conveyor) -> B_F_SORT/1
  Feedback5/2(F_62_P1) -> B_F_SORT/2
  Feedback5/3(F_62_P2) -> B_F_SORT/3
  Feedback5/4(F_62_Identify) -> B_F_SORT/4
  Feedback5/5(F_63_Led_Start) -> B_F_SORT/5
  Feedback5/6(F_63_Led_Reset) -> B_F_SORT/6
  Feedback5/7(F_63_Led_Extra1) -> B_F_SORT/7
  Feedback5/8(F_63_Led_Extra2) -> B_F_SORT/8
  Feedback5/9(F_63_Panel_O4) -> B_F_SORT/9
  Feedback5/10(F_63_Panel_O5) -> B_F_SORT/10
  Feedback5/11(F_63_Panel_O6) -> B_F_SORT/11
  Feedback5/12(F_63_Panel_O7) -> B_F_SORT/12
  Sensors5/1(O_60_SPart) -> B_S_SORT/1
  Sensors5/2(O_60_Slnd) -> B_S_SORT/2
  Sensors5/3(O_60_SPhoto) -> B_S_SORT/3
  Sensors5/4(O_60_Part_Pass) -> B_S_SORT/4
  Sensors5/5(O_60_SL1_Bck) -> B_S_SORT/5
  Sensors5/6(O_60_SL1_Fwd) -> B_S_SORT/6
  Sensors5/7(O_60_SL2_Bck) -> B_S_SORT/7
  Sensors5/8(O_60_SL2_Fwd) -> B_S_SORT/8
  Sensors5/9(O_61_Start) -> B_S_SORT/9
  Sensors5/10(O_61_Stop) -> B_S_SORT/10
  Sensors5/11(O_61_Key_Pos) -> B_S_SORT/11
  Sensors5/12(O_61_Reset) -> B_S_SORT/12
  Sensors5/13(O_61_Panel_I4) -> B_S_SORT/13
  Sensors5/14(O_61_Panel_I5) -> B_S_SORT/14
  Sensors5/15(O_61_Panel_I6) -> B_S_SORT/15
  Sensors5/16(O_61_Panel_I7) -> B_S_SORT/16
  B_C_SORT/1 -> Chart/21(Control_60)
  B_F_SORT/1 -> Chart/15(Actuators_60)
  B_S_SORT/1 -> Chart/27(Sensors_60)
  MATLAB Function1/1(C_45_Initialization) -> B_C_STORAGE/1
  MATLAB Function1/2(C_42_Profibus) -> B_C_STORAGE/2
  MATLAB Function1/3(C_45_Start) -> B_C_STORAGE/3
  MATLAB Function1/4(C_45_StorePart) -> B_C_STORAGE/4
  MATLAB Function1/5(C_45_RetrievePart) -> B_C_STORAGE/5
  MATLAB Function2/1(F_43_Led_Start) -> B_F_STORAGE/1
  MATLAB Function2/2(F_43_Led_Reset) -> B_F_STORAGE/2
  MATLAB Function2/3(F_43_Led_Extra1) -> B_F_STORAGE/3
  MATLAB Function2/4(F_43_Led_Extra2) -> B_F_STORAGE/4
  MATLAB Function2/5(F_43_Panel_O4) -> B_F_STORAGE/5
  MATLAB Function2/6(F_43_Panel_O5) -> B_F_STORAGE/6
  MATLAB Function2/7(F_43_Panel_O6) -> B_F_STORAGE/7
  MATLAB Function2/8(F_43_Panel_O7) -> B_F_STORAGE/8
  MATLAB Function3/1(O_41_Start) -> B_S_STORAGE/1
  MATLAB Function3/2(O_41_Stop) -> B_S_STORAGE/2
  MATLAB Function3/3(O_41_Key_Pos) -> B_S_STORAGE/3
  MATLAB Function3/4(O_41_Reset) -> B_S_STORAGE/4
  MATLAB Function3/5(O_41_Panel_I4) -> B_S_STORAGE/5
  MATLAB Function3/6(O_41_Panel_I5) -> B_S_STORAGE/6
  MATLAB Function3/7(O_41_Panel_I6) -> B_S_STORAGE/7
  MATLAB Function3/8(O_41_Panel_I7) -> B_S_STORAGE/8
  B_ASI_STORAGE/1 -> Chart/30(AS_i_40)
  B_C_STORAGE/1 -> Chart/29(Control_40)
  B_F_STORAGE/1 -> Chart/31(Actuators_40)
  B_S_STORAGE/1 -> Chart/32(Sensors_40)
  controls/1(C_85_Initialization) -> B_C_DIST/1
  controls/2(C_85_Part_Del) -> B_C_DIST/2
  controls/3(C_85_Part_Mag) -> B_C_DIST/3
  controls/4(C_86_Mag_Parts) -> B_C_DIST/4
  controls/5(C_87_RQ_MParts) -> B_C_DIST/5
  controls/6(C_82_Profibus) -> B_C_DIST/6
  controls/7(C_83_RQ_Parts) -> B_C_DIST/7
  controls/8(C_85_Start) -> B_C_DIST/8
  controls/9(C_85_Single) -> B_C_DIST/9
  controls/10(C_85_Continuous) -> B_C_DIST/10
  controls/11(C_85_Counted) -> B_C_DIST/11
  Asi/1(A_54_Request) -> B_ASI_HD1/1
  Asi/2(A_54_No_Cart) -> B_ASI_HD1/2
  Asi/3(A_54_Cart_Full) -> B_ASI_HD1/3
  Asi/4(A_54_CRoute_Out) -> B_ASI_HD1/4
  Asi/5(A_53_SortCartID) -> B_ASI_HD1/5
  Asi/6(A_54_Cart_Stat) -> B_ASI_HD1/6
  Asi/7(A_54_Cart_Next) -> B_ASI_HD1/7
  Asi/8(A_54_Optic) -> B_ASI_HD1/8
  Asi/9(A_54_Count) -> B_ASI_HD1/9
  Asi/10(A_54_Pist_Bck) -> B_ASI_HD1/10
  Asi/11(A_54_Release_FB) -> B_ASI_HD1/11
  Asi/12(A_54_CRoute_In) -> B_ASI_HD1/12
  fcn_Control_ROBOT/1(C_35_Part_Del) -> B_C_ROBOT/1
  fcn_Control_ROBOT/2(C_30_Robot1) -> B_C_ROBOT/2
  fcn_Control_ROBOT/3(C_30_Robot2) -> B_C_ROBOT/3
  fcn Asi Storage/1(A_44_Request) -> B_ASI_STORAGE/1
  fcn Asi Storage/2(A_44_No_Cart) -> B_ASI_STORAGE/2
  fcn Asi Storage/3(A_44_Cart_Full) -> B_ASI_STORAGE/3
  fcn Asi Storage/4(A_44_CRoute_In) -> B_ASI_STORAGE/4
  fcn Asi Storage/5(A_43_StorCartID) -> B_ASI_STORAGE/5
  fcn Asi Storage/6(A_44_Cart_Stat) -> B_ASI_STORAGE/6
  fcn Asi Storage/7(A_44_Cart_Next) -> B_ASI_STORAGE/7
  fcn Asi Storage/8(A_44_Optic) -> B_ASI_STORAGE/8
  fcn Asi Storage/9(A_44_Count) -> B_ASI_STORAGE/9
  fcn Asi Storage/10(A_44_Pist_Bck) -> B_ASI_STORAGE/10
  fcn Asi Storage/11(A_44_Release_FB) -> B_ASI_STORAGE/11
  fcn Asi Storage/12(A_44_CRoute_Out) -> B_ASI_STORAGE/12
  OPC UA Read6/1 -> Bus Selector/1, Bus Selector1/1, Bus Selector2/1, Bus Selector7/1, Bus Selector6/1, Bus Selector5/1, Bus Selector4/1, Bus Selector3/1
  Bus Selector/1 -> fcn Asi Storage/1(u1)  "<Value_2551>"
  Bus Selector/2 -> fcn Asi Storage/2(u2)  "<Value_2561>"
  Bus Selector/3 -> fcn Asi Storage/3(u3)  "<Value_2571>"
  Bus Selector/4 -> fcn Asi Storage/4(u4)  "<Value_2581>"
  Bus Selector/5 -> fcn Asi Storage/5(u5)  "<Value_2591>"
  Bus Selector/6 -> fcn Asi Storage/6(u6)  "<Value_2601>"
  Bus Selector/7 -> fcn Asi Storage/7(u7)  "<Value_2611>"
  Bus Selector/8 -> fcn Asi Storage/8(u8)  "<Value_2621>"
  Bus Selector/9 -> fcn Asi Storage/9(u9)  "<Value_2631>"
  Bus Selector/10 -> fcn Asi Storage/10(u10)  "<Value_2641>"
  Bus Selector/11 -> fcn Asi Storage/11(u11)  "<Value_2651>"
  Bus Selector/12 -> fcn Asi Storage/12(u12)  "<Value_2661>"
  Bus Selector1/1 -> MATLAB Function1/1(u1)  "<Value_2677>"
  Bus Selector1/2 -> MATLAB Function1/2(u2)  "<Value_2687>"
  Bus Selector1/3 -> MATLAB Function1/3(u3)  "<Value_2697>"
  Bus Selector1/4 -> MATLAB Function1/4(u4)  "<Value_2707>"
  Bus Selector1/5 -> MATLAB Function1/5(u5)  "<Value_2717>"
  Bus Selector2/1 -> MATLAB Function2/1(u1)  "<Value_2733>"
  Bus Selector2/2 -> MATLAB Function2/2(u2)  "<Value_2743>"
  Bus Selector2/3 -> MATLAB Function2/3(u3)  "<Value_2753>"
  Bus Selector2/4 -> MATLAB Function2/4(u4)  "<Value_2763>"
  Bus Selector2/5 -> MATLAB Function2/5(u5)  "<Value_2773>"
  Bus Selector2/6 -> MATLAB Function2/6(u6)  "<Value_2783>"
  Bus Selector2/7 -> MATLAB Function2/7(u7)  "<Value_2793>"
  Bus Selector2/8 -> MATLAB Function2/8(u8)  "<Value_2803>"
  Bus Selector3/1 -> MATLAB Function3/1(u1)  "<Value_2822>"
  Bus Selector3/2 -> MATLAB Function3/2(u2)  "<Value_2835>"
  Bus Selector3/3 -> MATLAB Function3/3(u3)  "<Value_2848>"
  Bus Selector3/4 -> MATLAB Function3/4(u4)  "<Value_2861>"
  Bus Selector3/5 -> MATLAB Function3/5(u5)  "<Value_2874>"
  Bus Selector3/6 -> MATLAB Function3/6(u6)  "<Value_2887>"
  Bus Selector3/7 -> MATLAB Function3/7(u7)  "<Value_2900>"
  Bus Selector3/8 -> MATLAB Function3/8(u8)  "<Value_2913>"
  Bus Selector4/1 -> fcn_Asi_ROBOT/1(u1)  "<Value_1245>"
  Bus Selector4/2 -> fcn_Asi_ROBOT/2(u2)  "<Value_1255>"
  Bus Selector4/3 -> fcn_Asi_ROBOT/3(u3)  "<Value_1265>"
  Bus Selector4/4 -> fcn_Asi_ROBOT/4(u4)  "<Value_1275>"
  Bus Selector4/5 -> fcn_Asi_ROBOT/5(u5)  "<Value_1285>"
  Bus Selector4/6 -> fcn_Asi_ROBOT/6(u6)  "<Value_1295>"
  Bus Selector4/7 -> fcn_Asi_ROBOT/7(u7)  "<Value_1305>"
  Bus Selector4/8 -> fcn_Asi_ROBOT/8(u8)  "<Value_1315>"
  Bus Selector4/9 -> fcn_Asi_ROBOT/9(u9)  "<Value_1325>"
  Bus Selector4/10 -> fcn_Asi_ROBOT/10(u10)  "<Value_1335>"
  Bus Selector4/11 -> fcn_Asi_ROBOT/11(u11)  "<Value_1345>"
  Bus Selector4/12 -> fcn_Asi_ROBOT/12(u12)  "<Value_1355>"
  Bus Selector5/1 -> fcn_Control_ROBOT/1(u1)  "<Value_1371>"
  Bus Selector5/2 -> fcn_Control_ROBOT/2(u2)  "<Value_1384>"
  Bus Selector5/3 -> fcn_Control_ROBOT/3(u3)  "<Value_1397>"
  Bus Selector6/1 -> fcn_Feedback_ROBOT/1(u1)  "<Value_1413>"
  Bus Selector6/2 -> fcn_Feedback_ROBOT/2(u2)  "<Value_1423>"
  Bus Selector6/3 -> fcn_Feedback_ROBOT/3(u3)  "<Value_1433>"
  Bus Selector6/4 -> fcn_Feedback_ROBOT/4(u4)  "<Value_1443>"
  Bus Selector6/5 -> fcn_Feedback_ROBOT/5(u5)  "<Value_1453>"
  Bus Selector6/6 -> fcn_Feedback_ROBOT/6(u6)  "<Value_1463>"
  Bus Selector7/1 -> fcn_Sensors_ROBOT/1(u1)  "<Value_1599>"
  Bus Selector7/2 -> fcn_Sensors_ROBOT/2(u2)  "<Value_1612>"
  Bus Selector7/3 -> fcn_Sensors_ROBOT/3(u3)  "<Value_1625>"
  Bus Selector7/4 -> fcn_Sensors_ROBOT/4(u4)  "<Value_1638>"
  Bus Selector7/5 -> fcn_Sensors_ROBOT/5(u5)  "<Value_1651>"
  Bus Selector7/6 -> fcn_Sensors_ROBOT/6(u6)  "<Value_1664>"
  Bus Selector7/7 -> fcn_Sensors_ROBOT/7(u7)  "<Value_1677>"
  Bus Selector7/8 -> fcn_Sensors_ROBOT/8(u8)  "<Value_1690>"
  Bus Selector7/9 -> fcn_Sensors_ROBOT/9(u9)  "<Value_1703>"
  Bus Selector7/10 -> fcn_Sensors_ROBOT/10(u10)  "<Value_1716>"
  Bus Selector7/11 -> fcn_Sensors_ROBOT/11(u11)  "<Value_1729>"
  Bus Selector7/12 -> fcn_Sensors_ROBOT/12(u12)  "<Value_1742>"
  OPC UA Read4/1 -> Bus Selector11/1, Bus Selector10/1, Bus Selector8/1, Bus Selector9/1
  Bus Selector8/1 -> Asi1_HAND2/1(u1)  "<Value_1176>"
  Bus Selector8/2 -> Asi1_HAND2/2(u2)  "<Value_1186>"
  Bus Selector8/3 -> Asi1_HAND2/3(u3)  "<Value_1196>"
  Bus Selector8/4 -> Asi1_HAND2/4(u4)  "<Value_1206>"
  Bus Selector8/5 -> Asi1_HAND2/5(u5)  "<Value_1216>"
  Bus Selector8/6 -> Asi1_HAND2/6(u6)  "<Value_1226>"
  Bus Selector8/7 -> Asi1_HAND2/7(u7)  "<Value_1236>"
  Bus Selector8/8 -> Asi1_HAND2/8(u8)  "<Value_1246>"
  Bus Selector8/9 -> Asi1_HAND2/9(u9)  "<Value_1256>"
  Bus Selector8/10 -> Asi1_HAND2/10(u10)  "<Value_1266>"
  Bus Selector8/11 -> Asi1_HAND2/11(u11)  "<Value_1276>"
  Bus Selector8/12 -> Asi1_HAND2/12(u12)  "<Value_1286>"
  Bus Selector9/1 -> Control3/1(u1)  "<Value_1302>"
  Bus Selector9/2 -> Control3/2(u2)  "<Value_1312>"
  Bus Selector9/3 -> Control3/3(u3)  "<Value_1322>"
  Bus Selector9/4 -> Control3/4(u4)  "<Value_1332>"
  Bus Selector9/5 -> Control3/5(u5)  "<Value_1342>"
  Bus Selector9/6 -> Control3/6(u6)  "<Value_1352>"
  Bus Selector9/7 -> Control3/7(u7)  "<Value_1362>"
  Bus Selector10/1 -> Feedback3/1(u1)  "<Value_1378>"
  Bus Selector10/2 -> Feedback3/2(u2)  "<Value_1388>"
  Bus Selector10/3 -> Feedback3/3(u3)  "<Value_1398>"
  Bus Selector10/4 -> Feedback3/4(u4)  "<Value_1408>"
  Bus Selector10/5 -> Feedback3/5(u5)  "<Value_1418>"
  Bus Selector10/6 -> Feedback3/6(u6)  "<Value_1428>"
  Bus Selector10/7 -> Feedback3/7(u7)  "<Value_1438>"
  Bus Selector10/8 -> Feedback3/8(u8)  "<Value_1448>"
  Bus Selector10/9 -> Feedback3/9(u9)  "<Value_1458>"
  Bus Selector10/10 -> Feedback3/10(u10)  "<Value_1468>"
  Bus Selector10/11 -> Feedback3/11(u11)  "<Value_1478>"
  Bus Selector10/12 -> Feedback3/12(u12)  "<Value_1488>"
  Bus Selector11/1 -> Sensors3/1(u1)  "<Value_1509>"
  Bus Selector11/2 -> Sensors3/2(u2)  "<Value_1522>"
  Bus Selector11/3 -> Sensors3/3(u3)  "<Value_1537>"
  Bus Selector11/4 -> Sensors3/4(u4)  "<Value_1550>"
  Bus Selector11/5 -> Sensors3/5(u5)  "<Value_1563>"
  Bus Selector11/6 -> Sensors3/6(u6)  "<Value_1576>"
  Bus Selector11/7 -> Sensors3/7(u7)  "<Value_1589>"
  Bus Selector11/8 -> Sensors3/8(u8)  "<Value_1602>"
  Bus Selector11/9 -> Sensors3/9(u9)  "<Value_1615>"
  Bus Selector11/10 -> Sensors3/10(u10)  "<Value_1628>"
  Bus Selector11/11 -> Sensors3/11(u11)  "<Value_1641>"
  Bus Selector11/12 -> Sensors3/12(u12)  "<Value_1654>"
  Bus Selector11/13 -> Sensors3/13(u13)  "<Value_1667>"
  Bus Selector11/14 -> Sensors3/14(u14)  "<Value_1680>"
  Bus Selector11/15 -> Sensors3/15(u15)  "<Value_1693>"
  OPC UA Read3/1 -> Bus Selector15/1, Bus Selector14/1, Bus Selector12/1, Bus Selector13/1
  Bus Selector12/1 -> Asi/1(u1)  "<Value_1457>"
  Bus Selector12/2 -> Asi/2(u2)  "<Value_1467>"
  Bus Selector12/3 -> Asi/3(u3)  "<Value_1477>"
  Bus Selector12/4 -> Asi/4(u4)  "<Value_1487>"
  Bus Selector12/5 -> Asi/5(u5)  "<Value_1497>"
  Bus Selector12/6 -> Asi/6(u6)  "<Value_1507>"
  Bus Selector12/7 -> Asi/7(u7)  "<Value_1517>"
  Bus Selector12/8 -> Asi/8(u8)  "<Value_1527>"
  Bus Selector12/9 -> Asi/9(u9)  "<Value_1537>"
  Bus Selector12/10 -> Asi/10(u10)  "<Value_1547>"
  Bus Selector12/11 -> Asi/11(u11)  "<Value_1557>"
  Bus Selector12/12 -> Asi/12(u12)  "<Value_1567>"
  Bus Selector13/1 -> Control2/1(u1)  "<Value_1583>"
  Bus Selector13/2 -> Control2/2(u2)  "<Value_1593>"
  Bus Selector13/3 -> Control2/3(u3)  "<Value_1603>"
  Bus Selector13/4 -> Control2/4(u4)  "<Value_1613>"
  Bus Selector13/5 -> Control2/5(u5)  "<Value_1623>"
  Bus Selector14/1 -> Feedback2/1(u1)  "<Value_1639>"
  Bus Selector14/2 -> Feedback2/2(u2)  "<Value_1649>"
  Bus Selector14/3 -> Feedback2/3(u3)  "<Value_1659>"
  Bus Selector14/4 -> Feedback2/4(u4)  "<Value_1669>"
  Bus Selector14/5 -> Feedback2/5(u5)  "<Value_1679>"
  Bus Selector14/6 -> Feedback2/6(u6)  "<Value_1689>"
  Bus Selector14/7 -> Feedback2/7(u7)  "<Value_1699>"
  Bus Selector14/8 -> Feedback2/8(u8)  "<Value_1709>"
  Bus Selector14/9 -> Feedback2/9(u9)  "<Value_1719>"
  Bus Selector14/10 -> Feedback2/10(u10)  "<Value_1729>"
  Bus Selector14/11 -> Feedback2/11(u11)  "<Value_1739>"
  Bus Selector14/12 -> Feedback2/12(u12)  "<Value_1749>"
  Bus Selector15/1 -> Sensors2/1(u1)  "<Value_1768>"
  Bus Selector15/2 -> Sensors2/2(u2)  "<Value_1781>"
  Bus Selector15/3 -> Sensors2/3(u3)  "<Value_1796>"
  Bus Selector15/4 -> Sensors2/4(u4)  "<Value_1809>"
  Bus Selector15/5 -> Sensors2/5(u5)  "<Value_1822>"
  Bus Selector15/6 -> Sensors2/6(u6)  "<Value_1835>"
  Bus Selector15/7 -> Sensors2/7(u7)  "<Value_1848>"
  Bus Selector15/8 -> Sensors2/8(u8)  "<Value_1861>"
  Bus Selector15/9 -> Sensors2/9(u9)  "<Value_1874>"
  Bus Selector15/10 -> Sensors2/10(u10)  "<Value_1887>"
  Bus Selector15/11 -> Sensors2/11(u11)  "<Value_1900>"
  Bus Selector15/12 -> Sensors2/12(u12)  "<Value_1913>"
  Bus Selector15/13 -> Sensors2/13(u13)  "<Value_1926>"
  Bus Selector15/14 -> Sensors2/14(u14)  "<Value_1939>"
  Bus Selector15/15 -> Sensors2/15(u15)  "<Value_1952>"
  OPC UA Read/1 -> Bus Selector18/1, Bus Selector17/1, Bus Selector16/1
  Bus Selector16/1 -> controls/1(u1)  "<Value_1195>"
  Bus Selector16/2 -> controls/2(u2)  "<Value_1205>"
  Bus Selector16/3 -> controls/3(u3)  "<Value_1215>"
  Bus Selector16/4 -> controls/4(u4)  "<Value_1227>"
  Bus Selector16/5 -> controls/5(u5)  "<Value_1239>"
  Bus Selector16/6 -> controls/6(u6)  "<Value_1249>"
  Bus Selector16/7 -> controls/7(u7)  "<Value_1261>"
  Bus Selector16/8 -> controls/8(u8)  "<Value_1271>"
  Bus Selector16/9 -> controls/9(u9)  "<Value_1281>"
  Bus Selector16/10 -> controls/10(u10)  "<Value_1291>"
  Bus Selector16/11 -> controls/11(u11)  "<Value_1301>"
  Bus Selector17/1 -> feedback/1(u1)  "<Value_1317>"
  Bus Selector17/2 -> feedback/2(u2)  "<Value_1327>"
  Bus Selector17/3 -> feedback/3(u3)  "<Value_1337>"
  Bus Selector17/4 -> feedback/4(u4)  "<Value_1347>"
  Bus Selector17/5 -> feedback/5(u5)  "<Value_1357>"
  Bus Selector17/6 -> feedback/6(u6)  "<Value_1367>"
  Bus Selector17/7 -> feedback/7(u7)  "<Value_1377>"
  Bus Selector17/8 -> feedback/8(u8)  "<Value_1387>"
  Bus Selector17/9 -> feedback/9(u9)  "<Value_1397>"
  Bus Selector17/10 -> feedback/10(u10)  "<Value_1407>"
  Bus Selector17/11 -> feedback/11(u11)  "<Value_1417>"
  Bus Selector17/12 -> feedback/12(u12)  "<Value_1427>"
  Bus Selector17/13 -> feedback/13(u13)  "<Value_1437>"
  Bus Selector18/1 -> sensors/1(u1)  "<Value_1458>"
  Bus Selector18/2 -> sensors/2(u2)  "<Value_1471>"
  Bus Selector18/3 -> sensors/3(u3)  "<Value_1486>"
  Bus Selector18/4 -> sensors/4(u4)  "<Value_1499>"
  Bus Selector18/5 -> sensors/5(u5)  "<Value_1512>"
  Bus Selector18/6 -> sensors/6(u6)  "<Value_1525>"
  Bus Selector18/7 -> sensors/7(u7)  "<Value_1538>"
  Bus Selector18/8 -> sensors/8(u8)  "<Value_1551>"
  Bus Selector18/9 -> sensors/9(u9)  "<Value_1564>"
  Bus Selector18/10 -> sensors/10(u10)  "<Value_1577>"
  Bus Selector18/11 -> sensors/11(u11)  "<Value_1590>"
  Bus Selector18/12 -> sensors/12(u12)  "<Value_1603>"
  Bus Selector18/13 -> sensors/13(u13)  "<Value_1616>"
  Bus Selector18/14 -> sensors/14(u14)  "<Value_1629>"
  Bus Selector18/15 -> sensors/15(u15)  "<Value_1642>"
  OPC UA Read1/1 -> Bus Selector22/1, Bus Selector21/1, Bus Selector19/1, Bus Selector20/1
  Bus Selector19/1 -> ASI/1(u1)  "<Value_1455>"
  Bus Selector19/2 -> ASI/2(u2)  "<Value_1465>"
  Bus Selector19/3 -> ASI/3(u3)  "<Value_1475>"
  Bus Selector19/4 -> ASI/4(u4)  "<Value_1485>"
  Bus Selector19/5 -> ASI/5(u5)  "<Value_1495>"
  Bus Selector19/6 -> ASI/6(u6)  "<Value_1505>"
  Bus Selector19/7 -> ASI/7(u7)  "<Value_1515>"
  Bus Selector19/8 -> ASI/8(u8)  "<Value_1525>"
  Bus Selector19/9 -> ASI/9(u9)  "<Value_1535>"
  Bus Selector19/10 -> ASI/10(u10)  "<Value_1545>"
  Bus Selector19/11 -> ASI/11(u11)  "<Value_1555>"
  Bus Selector19/12 -> ASI/12(u12)  "<Value_1565>"
  Bus Selector19/13 -> ASI/13(u13)  "<Value_1575>"
  Bus Selector20/1 -> Control/1(u1)  "<Value_1591>"
  Bus Selector20/2 -> Control/2(u2)  "<Value_1601>"
  Bus Selector20/3 -> Control/3(u3)  "<Value_1611>"
  Bus Selector20/4 -> Control/4(u4)  "<Value_1621>"
  Bus Selector20/5 -> Control/5(u5)  "<Value_1631>"
  Bus Selector20/6 -> Control/6(u6)  "<Value_1641>"
  Bus Selector20/7 -> Control/7(u7)  "<Value_1651>"
  Bus Selector20/8 -> Control/8(u8)  "<Value_1661>"
  Bus Selector20/9 -> Control/9(u9)  "<Value_1671>"
  Bus Selector20/10 -> Control/10(u10)  "<Value_1681>"
  Bus Selector20/11 -> Control/11(u11)  "<Value_1691>"
  Bus Selector20/12 -> Control/12(u12)  "<Value_1701>"
  Bus Selector20/13 -> Control/13(u13)  "<Value_1711>"
  Bus Selector21/1 -> Feedback/1(u1)  "<Value_1727>"
  Bus Selector21/2 -> Feedback/2(u2)  "<Value_1737>"
  Bus Selector21/3 -> Feedback/3(u3)  "<Value_1747>"
  Bus Selector21/4 -> Feedback/4(u4)  "<Value_1757>"
  Bus Selector21/5 -> Feedback/5(u5)  "<Value_1767>"
  Bus Selector21/6 -> Feedback/6(u6)  "<Value_1777>"
  Bus Selector21/7 -> Feedback/7(u7)  "<Value_1787>"
  Bus Selector21/8 -> Feedback/8(u8)  "<Value_1797>"
  Bus Selector21/9 -> Feedback/9(u9)  "<Value_1807>"
  Bus Selector21/10 -> Feedback/10(u10)  "<Value_1817>"
  Bus Selector21/11 -> Feedback/11(u11)  "<Value_1827>"
  Bus Selector21/12 -> Feedback/12(u12)  "<Value_1837>"
  Bus Selector22/1 -> Sensors/1(u1)  "<Value_1858>"
  Bus Selector22/2 -> Sensors/2(u2)  "<Value_1871>"
  Bus Selector22/3 -> Sensors/3(u3)  "<Value_1886>"
  Bus Selector22/4 -> Sensors/4(u4)  "<Value_1899>"
  Bus Selector22/5 -> Sensors/5(u5)  "<Value_1912>"
  Bus Selector22/6 -> Sensors/6(u6)  "<Value_1925>"
  Bus Selector22/7 -> Sensors/7(u7)  "<Value_1938>"
  Bus Selector22/8 -> Sensors/8(u8)  "<Value_1951>"
  Bus Selector22/9 -> Sensors/9(u9)  "<Value_1964>"
  Bus Selector22/10 -> Sensors/10(u10)  "<Value_1977>"
  Bus Selector22/11 -> Sensors/11(u11)  "<Value_1990>"
  Bus Selector22/12 -> Sensors/12(u12)  "<Value_2003>"
  Bus Selector22/13 -> Sensors/13(u13)  "<Value_2016>"
  Bus Selector22/14 -> Sensors/14(u14)  "<Value_2029>"
  Bus Selector22/15 -> Sensors/15(u15)  "<Value_2042>"
  OPC UA Read2/1 -> Bus Selector25/1, Bus Selector24/1, Bus Selector23/1
  Bus Selector23/1 -> Control1/1(u1)  "<Value_1382>"
  Bus Selector23/2 -> Control1/2(u2)  "<Value_1392>"
  Bus Selector23/3 -> Control1/3(u3)  "<Value_1402>"
  Bus Selector23/4 -> Control1/4(u4)  "<Value_1412>"
  Bus Selector23/5 -> Control1/5(u5)  "<Value_1422>"
  Bus Selector23/6 -> Control1/6(u6)  "<Value_1432>"
  Bus Selector23/7 -> Control1/7(u7)  "<Value_1442>"
  Bus Selector23/8 -> Control1/8(u8)  "<Value_1452>"
  Bus Selector23/9 -> Control1/9(u9)  "<Value_1462>"
  Bus Selector23/10 -> Control1/10(u10)  "<Value_1472>"
  Bus Selector23/11 -> Control1/11(u11)  "<Value_1482>"
  Bus Selector23/12 -> Control1/12(u12)  "<Value_1492>"
  Bus Selector23/13 -> Control1/13(u13)  "<Value_1502>"
  Bus Selector23/14 -> Control1/14(u14)  "<Value_1512>"
  Bus Selector23/15 -> Control1/15(u15)  "<Value_1522>"
  Bus Selector23/16 -> Control1/16(u16)  "<Value_1532>"
  Bus Selector23/17 -> Control1/17(u17)  "<Value_1542>"
  Bus Selector23/18 -> Control1/18(u18)  "<Value_1552>"
  Bus Selector23/19 -> Control1/19(u19)  "<Value_1562>"
  Bus Selector23/20 -> Control1/20(u20)  "<Value_1572>"
  Bus Selector23/21 -> Control1/21(u21)  "<Value_1582>"
  Bus Selector23/22 -> Control1/22(u22)  "<Value_1592>"
  Bus Selector23/23 -> Control1/23(u23)  "<Value_1602>"
  Bus Selector23/24 -> Control1/24(u24)  "<Value_1612>"
  Bus Selector24/1 -> Feedback1/1(u1)  "<Value_1628>"
  Bus Selector24/2 -> Feedback1/2(u2)  "<Value_1638>"
  Bus Selector24/3 -> Feedback1/3(u3)  "<Value_1648>"
  Bus Selector24/4 -> Feedback1/4(u4)  "<Value_1658>"
  Bus Selector24/5 -> Feedback1/5(u5)  "<Value_1668>"
  Bus Selector24/6 -> Feedback1/6(u6)  "<Value_1678>"
  Bus Selector24/7 -> Feedback1/7(u7)  "<Value_1688>"
  Bus Selector24/8 -> Feedback1/8(u8)  "<Value_1698>"
  Bus Selector24/9 -> Feedback1/9(u9)  "<Value_1708>"
  Bus Selector25/1 -> Sensors1/1(u1)  "<Value_1727>"
  Bus Selector25/2 -> Sensors1/2(u2)  "<Value_1740>"
  Bus Selector25/3 -> Sensors1/3(u3)  "<Value_1755>"
  Bus Selector25/4 -> Sensors1/4(u4)  "<Value_1768>"
  Bus Selector25/5 -> Sensors1/5(u5)  "<Value_1781>"
  Bus Selector25/6 -> Sensors1/6(u6)  "<Value_1794>"
  Bus Selector25/7 -> Sensors1/7(u7)  "<Value_1807>"
  Bus Selector25/8 -> Sensors1/8(u8)  "<Value_1820>"
  Bus Selector25/9 -> Sensors1/9(u9)  "<Value_1833>"
  Bus Selector25/10 -> Sensors1/10(u10)  "<Value_1846>"
  Bus Selector25/11 -> Sensors1/11(u11)  "<Value_1859>"
  Bus Selector25/12 -> Sensors1/12(u12)  "<Value_1872>"
  Bus Selector25/13 -> Sensors1/13(u13)  "<Value_1885>"
  Bus Selector25/14 -> Sensors1/14(u14)  "<Value_1898>"
  Bus Selector25/15 -> Sensors1/15(u15)  "<Value_1911>"
  Bus Selector25/16 -> Sensors1/16(u16)  "<Value_1924>"
  Bus Selector25/17 -> Sensors1/17(u17)  "<Value_1937>"
  Bus Selector25/18 -> Sensors1/18(u18)  "<Value_1950>"
  Bus Selector25/19 -> Sensors1/19(u19)  "<Value_1963>"
  Bus Selector25/20 -> Sensors1/20(u20)  "<Value_1976>"
  Bus Selector25/21 -> Sensors1/21(u21)  "<Value_1989>"
  Bus Selector25/22 -> Sensors1/22(u22)  "<Value_2002>"
  Bus Selector25/23 -> Sensors1/23(u23)  "<Value_2015>"
  Bus Selector25/24 -> Sensors1/24(u24)  "<Value_2028>"
  Bus Selector25/25 -> Sensors1/25(u25)  "<Value_2041>"
  Bus Selector25/26 -> Sensors1/26(u26)  "<Value_2054>"
  Bus Selector25/27 -> Sensors1/27(u27)  "<Value_2067>"
  Bus Selector25/28 -> Sensors1/28(u28)  "<Value_2080>"
  Bus Selector25/29 -> Sensors1/29(u29)  "<Value_2093>"
  Bus Selector25/30 -> Sensors1/30(u30)  "<Value_2106>"
  Bus Selector25/31 -> Sensors1/31(u31)  "<Value_2119>"
  Bus Selector25/32 -> Sensors1/32(u32)  "<Value_2132>"
  Bus Selector25/33 -> Sensors1/33(u33)  "<Value_2145>"
  OPC UA Read5/1 -> Bus Selector28/1, Bus Selector27/1, Bus Selector26/1
  Bus Selector26/1 -> Control4/1(u1)  "<Value_1204>"
  Bus Selector26/2 -> Control4/2(u2)  "<Value_1214>"
  Bus Selector26/3 -> Control4/3(u3)  "<Value_1224>"
  Bus Selector26/4 -> Control4/4(u4)  "<Value_1234>"
  Bus Selector26/5 -> Control4/5(u5)  "<Value_1244>"
  Bus Selector26/6 -> Control4/6(u6)  "<Value_1254>"
  Bus Selector26/7 -> Control4/7(u7)  "<Value_1264>"
  Bus Selector26/8 -> Control4/8(u8)  "<Value_1274>"
  Bus Selector26/9 -> Control4/9(u9)  "<Value_1284>"
  Bus Selector26/10 -> Control4/10(u10)  "<Value_1294>"
  Bus Selector27/1 -> Feedback4/1(u1)  "<Value_1310>"
  Bus Selector27/2 -> Feedback4/2(u2)  "<Value_1320>"
  Bus Selector27/3 -> Feedback4/3(u3)  "<Value_1330>"
  Bus Selector27/4 -> Feedback4/4(u4)  "<Value_1340>"
  Bus Selector27/5 -> Feedback4/5(u5)  "<Value_1350>"
  Bus Selector27/6 -> Feedback4/6(u6)  "<Value_1360>"
  Bus Selector27/7 -> Feedback4/7(u7)  "<Value_1370>"
  Bus Selector27/8 -> Feedback4/8(u8)  "<Value_1380>"
  Bus Selector27/9 -> Feedback4/9(u9)  "<Value_1390>"
  Bus Selector27/10 -> Feedback4/10(u10)  "<Value_1400>"
  Bus Selector27/11 -> Feedback4/11(u11)  "<Value_1410>"
  Bus Selector27/12 -> Feedback4/12(u12)  "<Value_1420>"
  Bus Selector27/13 -> Feedback4/13(u13)  "<Value_1430>"
  Bus Selector27/14 -> Feedback4/14(u14)  "<Value_1440>"
  Bus Selector28/1 -> Sensors4/1(u1)  "<Value_1461>"
  Bus Selector28/2 -> Sensors4/2(u2)  "<Value_1474>"
  Bus Selector28/3 -> Sensors4/3(u3)  "<Value_1489>"
  Bus Selector28/4 -> Sensors4/4(u4)  "<Value_1502>"
  Bus Selector28/5 -> Sensors4/5(u5)  "<Value_1515>"
  Bus Selector28/6 -> Sensors4/6(u6)  "<Value_1528>"
  Bus Selector28/7 -> Sensors4/7(u7)  "<Value_1541>"
  Bus Selector28/8 -> Sensors4/8(u8)  "<Value_1554>"
  Bus Selector28/9 -> Sensors4/9(u9)  "<Value_1567>"
  Bus Selector28/10 -> Sensors4/10(u10)  "<Value_1580>"
  Bus Selector28/11 -> Sensors4/11(u11)  "<Value_1593>"
  Bus Selector28/12 -> Sensors4/12(u12)  "<Value_1606>"
  Bus Selector28/13 -> Sensors4/13(u13)  "<Value_1619>"
  Bus Selector28/14 -> Sensors4/14(u14)  "<Value_1632>"
  Bus Selector28/15 -> Sensors4/15(u15)  "<Value_1645>"
  OPC UA Read7/1 -> Bus Selector31/1, Bus Selector30/1, Bus Selector29/1
  Bus Selector29/1 -> Control5/1(u1)  "<Value_1178>"
  Bus Selector29/2 -> Control5/2(u2)  "<Value_1188>"
  Bus Selector29/3 -> Control5/3(u3)  "<Value_1198>"
  Bus Selector29/4 -> Control5/4(u4)  "<Value_1208>"
  Bus Selector29/5 -> Control5/5(u5)  "<Value_1218>"
  Bus Selector29/6 -> Control5/6(u6)  "<Value_1228>"
  Bus Selector29/7 -> Control5/7(u7)  "<Value_1238>"
  Bus Selector29/8 -> Control5/8(u8)  "<Value_1248>"
  Bus Selector29/9 -> Control5/9(u9)  "<Value_1258>"
  Bus Selector29/10 -> Control5/10(u10)  "<Value_1268>"
  Bus Selector29/11 -> Control5/11(u11)  "<Value_1278>"
  Bus Selector30/1 -> Feedback5/1(u1)  "<Value_1294>"
  Bus Selector30/2 -> Feedback5/2(u2)  "<Value_1304>"
  Bus Selector30/3 -> Feedback5/3(u3)  "<Value_1314>"
  Bus Selector30/4 -> Feedback5/4(u4)  "<Value_1324>"
  Bus Selector30/5 -> Feedback5/5(u5)  "<Value_1334>"
  Bus Selector30/6 -> Feedback5/6(u6)  "<Value_1344>"
  Bus Selector30/7 -> Feedback5/7(u7)  "<Value_1354>"
  Bus Selector30/8 -> Feedback5/8(u8)  "<Value_1364>"
  Bus Selector30/9 -> Feedback5/9(u9)  "<Value_1374>"
  Bus Selector30/10 -> Feedback5/10(u10)  "<Value_1384>"
  Bus Selector30/11 -> Feedback5/11(u11)  "<Value_1394>"
  Bus Selector30/12 -> Feedback5/12(u12)  "<Value_1404>"
  Bus Selector31/1 -> Sensors5/1(u1)  "<Value_1423>"
  Bus Selector31/2 -> Sensors5/2(u2)  "<Value_1436>"
  Bus Selector31/3 -> Sensors5/3(u3)  "<Value_1451>"
  Bus Selector31/4 -> Sensors5/4(u4)  "<Value_1464>"
  Bus Selector31/5 -> Sensors5/5(u5)  "<Value_1477>"
  Bus Selector31/6 -> Sensors5/6(u6)  "<Value_1490>"
  Bus Selector31/7 -> Sensors5/7(u7)  "<Value_1503>"
  Bus Selector31/8 -> Sensors5/8(u8)  "<Value_1516>"
  Bus Selector31/9 -> Sensors5/9(u9)  "<Value_1529>"
  Bus Selector31/10 -> Sensors5/10(u10)  "<Value_1542>"
  Bus Selector31/11 -> Sensors5/11(u11)  "<Value_1555>"
  Bus Selector31/12 -> Sensors5/12(u12)  "<Value_1568>"
  Bus Selector31/13 -> Sensors5/13(u13)  "<Value_1581>"
  Bus Selector31/14 -> Sensors5/14(u14)  "<Value_1594>"
  Bus Selector31/15 -> Sensors5/15(u15)  "<Value_1607>"
  Bus Selector31/16 -> Sensors5/16(u16)  "<Value_1620>"
